simulink model "Copy_of_NDI"  (R2024b)
settings: Solver=ode4  StartTime=0  StopTime=100  FixedStep=fcs.Ts  RelTol=1e-3
PreLoadFcn:
  | FlightPhase = 'FallingLeaf';
  | % FlightPhase = 'InAir';
  | % FlightPhase = 'TVC_h10000V617alpha2';
  | run('PreLoadFcn.m')
values from neighbouring files (symbols this model uses):
  ControlAllocation = 1    [PreLoadFcn.m]    (also in RunThis_ChiaWei.m = 4; RunThis_LM.m = 4; RunThis_Shao.m; RunThis_james.m = 10)
  DUmax = IN_MAT(k+4,1:m)'    [LP_def.m]    (also in LP_lift.m; LP_sig.m; LP_thrust.m; PreLoadFcn.m = [Aactuator.right_aileron.RateLimitUpper Aactuator.left_ailer)
  DUmin = IN_MAT(k+5,1:m)'    [LP_def.m]    (also in LP_lift.m; LP_sig.m; LP_thrust.m; PreLoadFcn.m = [Aactuator.right_aileron.RateLimitLower Aactuator.left_ailer)
  g = [ 0  0  32.17 ]    [PreLoadFcn.m]
  hground = 0    [PreLoadFcn.m]
  m = m1-1    [CGIwrap.m]    (also in DAISY_CHAINING.m; DA_Allocation.m; LP_BasicSolution.m; LP_def.m)
  Mode_deflection_aileron = 1    [PreLoadFcn.m]    (also in RunThis_ChiaWei.m; RunThis_Shao.m = 0)
  Mode_deflection_elevator = 1    [PreLoadFcn.m]    (also in RunThis_ChiaWei.m; RunThis_Shao.m = 0)
  Mode_deflection_rudder = 1    [PreLoadFcn.m]    (also in RunThis_ChiaWei.m; RunThis_Shao.m = 0)
  Mode_deflection_TVC_y = 1    [PreLoadFcn.m]    (also in RunThis_ChiaWei.m; RunThis_Shao.m = 2)
  Mode_deflection_TVC_z = 1    [PreLoadFcn.m]    (also in RunThis_ChiaWei.m; RunThis_Shao.m = 0)
  N = IN_MAT(k+7:k+15,1:m)    [CGIwrap.m]    (also in DAISY_CHAINING.m; PreLoadFcn.m = [ 1      0     0.25; RunThis_ChiaWei.m = [ 1      0     0.25; RunThis_LM.m = [ 1      0     0.25)
  Ninv_2nozzle = inv(diag([  1/21.5  1/21.5  1/25  1/25  1/30  1/15  1/15  1/15  1/15 ]))    [PreLoadFcn.m]
  Ninv_no_nozzle = diag([    21.5    21.5    25    25    30    0     0     0     0  ])    [PreLoadFcn.m]
  state0 = [IC.npos IC.epos IC.alt IC.q0 IC.q1 IC.q2 IC.q3  IC.p IC.q IC.r IC.alpha IC.beta IC.mu IC.Vt IC.chi IC.gamma]    [PreLoadFcn.m]
  Umax_2nozzle = [Aactuator.right_aileron.AngleLimitUpper  Aactuator.left_aileron.AngleLimitUpper  Aactuator.right_elevator.AngleLimitUpper Aactuator.left_elevator.AngleLimitUpper  Aactuator.rudder.AngleLimitUpper                  Aactuator.TVC_ry.AngleLimitUpper    Aactuator.TVC_rz.AngleLimitUpper  Aactuator.TVC_ly.AngleLimitUpper    Aactuator.TVC_lz.AngleLimitUpper]    [PreLoadFcn.m]
  Umax_no_nozzle = [Aactuator.right_aileron.AngleLimitUpper  Aactuator.left_aileron.AngleLimitUpper  Aactuator.right_elevator.AngleLimitUpper Aactuator.left_elevator.AngleLimitUpper  Aactuator.rudder.AngleLimitUpper                    0 0 0 0]    [PreLoadFcn.m]
  Umin_2nozzle = [Aactuator.aileron.AngleLimitLower  Aactuator.aileron.AngleLimitLower  Aactuator.elevator.AngleLimitLower Aactuator.elevator.AngleLimitLower  Aactuator.rudder.AngleLimitLower                  Aactuator.TVC_ry.AngleLimitLower    Aactuator.TVC_rz.AngleLimitLower Aactuator.TVC_ly.AngleLimitLower    Aactuator.TVC_lz.AngleLimitLower]    [PreLoadFcn.m]
  Umin_no_nozzle = [Aactuator.right_aileron.AngleLimitLower  Aactuator.left_aileron.AngleLimitLower  Aactuator.right_elevator.AngleLimitLower Aactuator.left_elevator.AngleLimitLower  Aactuator.rudder.AngleLimitLower                    0 0 0 0]    [PreLoadFcn.m]
undefined symbols (not defined in the file or in its folder): Aactuator, ac, AeroCoeff, EngineTable, F, fcs, ft, IC, kg, LandingGear, Light, MIL, PIController, s, Sensor, sigbuilder_block, slug, sysID_DAQ, sysID_OBES, WMM2020
libraries: aerolibconvert2 x31, slpidlib x11, simulink x6, sharedutil x4, aerolibatmos2 x3, aerolibwind2 x3, aerolibbdyn x3, aerolibgravity2 x2, sharedtransform x1
(part 6 of 14)

== system Copy_of_NDI/F-16 Vehicle Systems Model/Pilot commands storehouse/trun(deg) 初始高度10000ft 初始速度100ft//s攻角30度 ==
  Demux : Demux  Tag=STV Demux  Outputs=5
      settings: DisplayOption=none
  FromWs : FromWorkspace  Tag=STV FromWs  VariableName=tuvar
      SigBuilderData=|
      | common.afterFinalStr = 'Extrapolate'
      | common.sampleTime = 0
      | dataSet.timeRange = [0 20]
      | dataSet.name = 'Group 5'
      | sbobj.Groups.Name = 'Group 5'
      | sbobj.Groups.Signals(1).Name = 'mu'
      | sbobj.Groups.Signals(1).XData = [0 2 5.5 6.5 8.2 9.5 10 13 15 20]
      | sbobj.Groups.Signals(1).YData = [0 0 0 -80 -120 -120 -120 -70 -40 -10]
      | sbobj.Groups.Signals(2).Name = 'alpha'
      | sbobj.Groups.Signals(2).XData = [0 4 7.8 9.2 12.5 14 16 20]
      | sbobj.Groups.Signals(2).YData = [5 5 30 30 10 5 5 5]
      | sbobj.Groups.Signals(3).Name = 'beta'
      | sbobj.Groups.Signals(3).XData = [0 20]
      | sbobj.Groups.Signals(3).YData = [0 0]
      | sbobj.Groups.Signals(4).Name = 'speed brake'
      | sbobj.Groups.Signals(4).XData = [0 20]
      | sbobj.Groups.Signals(4).YData = [0 0]
      | sbobj.Groups.Signals(5).Name = 'LandingGear_down'
      | sbobj.Groups.Signals(5).XData = [0 20]
      | sbobj.Groups.Signals(5).YData = [1 1]
      | sbobj.Groups.TimeRange = [0 20]
  mu : Outport  Tag=STV Outport  VectorParamsAs1DForOutWhenUnconnected=off
  alpha : Outport  Tag=STV Outport  Port=2  VectorParamsAs1DForOutWhenUnconnected=off
  beta : Outport  Tag=STV Outport  Port=3  VectorParamsAs1DForOutWhenUnconnected=off
  speed brake : Outport  Tag=STV Outport  Port=4
  LandingGear_down : Outport  Tag=STV Outport  Port=5
  wires:
  Demux/5 -> LandingGear_down/1
  Demux/4 -> speed brake/1
  Demux/3 -> beta/1
  Demux/2 -> alpha/1
  Demux/1 -> mu/1
  FromWs/1 -> Demux/1

== system Copy_of_NDI/F-16 Vehicle Systems Model/Pilot commands storehouse/trun(deg) 初始高度10000ft 初始速度150ft//s攻角40度1 ==
  Demux : Demux  Tag=STV Demux  Outputs=5
      settings: DisplayOption=none
  FromWs : FromWorkspace  Tag=STV FromWs  VariableName=tuvar
      SigBuilderData=|
      | common.afterFinalStr = 'Extrapolate'
      | common.sampleTime = 0
      | dataSet.timeRange = [0 20]
      | dataSet.name = 'Group 5'
      | sbobj.Groups.Name = 'Group 5'
      | sbobj.Groups.Signals(1).Name = 'mu'
      | sbobj.Groups.Signals(1).XData = [0 2 5.5 7 8.7 10 11 13 15 20]
      | sbobj.Groups.Signals(1).YData = [0 0 -19.5 -60 -150 -150 -150 -70 -40 -10]
      | sbobj.Groups.Signals(2).Name = 'alpha'
      | sbobj.Groups.Signals(2).XData = [0 5 7.8 8.2 10 12.5 14 20]
      | sbobj.Groups.Signals(2).YData = [7 10 40 40 20 10.68 10 10]
      | sbobj.Groups.Signals(3).Name = 'beta'
      | sbobj.Groups.Signals(3).XData = [0 20]
      | sbobj.Groups.Signals(3).YData = [0 0]
      | sbobj.Groups.Signals(4).Name = 'speed brake'
      | sbobj.Groups.Signals(4).XData = [0 20]
      | sbobj.Groups.Signals(4).YData = [0 0]
      | sbobj.Groups.Signals(5).Name = 'LandingGear_down'
      | sbobj.Groups.Signals(5).XData = [0 20]
      | sbobj.Groups.Signals(5).YData = [1 1]
      | sbobj.Groups.TimeRange = [0 20]
  mu : Outport  Tag=STV Outport  VectorParamsAs1DForOutWhenUnconnected=off
  alpha : Outport  Tag=STV Outport  Port=2  VectorParamsAs1DForOutWhenUnconnected=off
  beta : Outport  Tag=STV Outport  Port=3  VectorParamsAs1DForOutWhenUnconnected=off
  speed brake : Outport  Tag=STV Outport  Port=4
  LandingGear_down : Outport  Tag=STV Outport  Port=5
  wires:
  Demux/5 -> LandingGear_down/1
  Demux/4 -> speed brake/1
  Demux/3 -> beta/1
  Demux/2 -> alpha/1
  Demux/1 -> mu/1
  FromWs/1 -> Demux/1

== system Copy_of_NDI/F-16 Vehicle Systems Model/Pilot commands storehouse/trun(deg) 初始高度10000ft 初始速度250ft//s攻角40度1 ==
  Demux : Demux  Tag=STV Demux  Outputs=5
      settings: DisplayOption=none
  FromWs : FromWorkspace  Tag=STV FromWs  VariableName=tuvar
      SigBuilderData=|
      | common.afterFinalStr = 'Extrapolate'
      | common.sampleTime = 0
      | dataSet.timeRange = [0 20]
      | dataSet.name = 'Group 5'
      | sbobj.Groups.Name = 'Group 5'
      | sbobj.Groups.Signals(1).Name = 'mu'
      | sbobj.Groups.Signals(1).XData = [0 2 5.5 7 8.7 8.7 10 11 13 15 20]
      | sbobj.Groups.Signals(1).YData = [0 0 -19.5 -122 -172 -170 -170 -170 -70 -40 -10]
      | sbobj.Groups.Signals(2).Name = 'alpha'
      | sbobj.Groups.Signals(2).XData = [0 5 7.8 8.2 10 12.5 14 20]
      | sbobj.Groups.Signals(2).YData = [7 10 40 40 20 10.68 10 10]
      | sbobj.Groups.Signals(3).Name = 'beta'
      | sbobj.Groups.Signals(3).XData = [0 20]
      | sbobj.Groups.Signals(3).YData = [0 0]
      | sbobj.Groups.Signals(4).Name = 'speed brake'
      | sbobj.Groups.Signals(4).XData = [0 20]
      | sbobj.Groups.Signals(4).YData = [0 0]
      | sbobj.Groups.Signals(5).Name = 'LandingGear_down'
      | sbobj.Groups.Signals(5).XData = [0 20]
      | sbobj.Groups.Signals(5).YData = [1 1]
      | sbobj.Groups.TimeRange = [0 20]
  mu : Outport  Tag=STV Outport  VectorParamsAs1DForOutWhenUnconnected=off
  alpha : Outport  Tag=STV Outport  Port=2  VectorParamsAs1DForOutWhenUnconnected=off
  beta : Outport  Tag=STV Outport  Port=3  VectorParamsAs1DForOutWhenUnconnected=off
  speed brake : Outport  Tag=STV Outport  Port=4
  LandingGear_down : Outport  Tag=STV Outport  Port=5
  wires:
  Demux/5 -> LandingGear_down/1
  Demux/4 -> speed brake/1
  Demux/3 -> beta/1
  Demux/2 -> alpha/1
  Demux/1 -> mu/1
  FromWs/1 -> Demux/1

== system Copy_of_NDI/F-16 Vehicle Systems Model/Pilot commands storehouse/trun(deg) 初始高度10000ft 初始速度350ft//s攻角40度 ==
  Demux : Demux  Tag=STV Demux  Outputs=5
      settings: DisplayOption=none
  FromWs : FromWorkspace  Tag=STV FromWs  VariableName=tuvar
      SigBuilderData=|
      | common.afterFinalStr = 'Extrapolate'
      | common.sampleTime = 0
      | dataSet.timeRange = [0 20]
      | dataSet.name = 'Group 5'
      | sbobj.Groups.Name = 'Group 5'
      | sbobj.Groups.Signals(1).Name = 'mu'
      | sbobj.Groups.Signals(1).XData = [0 2 5.5 6.5 8.2 10 11 13 15 20]
      | sbobj.Groups.Signals(1).YData = [0 0 -19.5 -122 -170 -170 -170 -70 -40 -10]
      | sbobj.Groups.Signals(2).Name = 'alpha'
      | sbobj.Groups.Signals(2).XData = [0 5 7.8 8.2 10 12.5 14 20]
      | sbobj.Groups.Signals(2).YData = [7 10 40 40 20 10.68 10 10]
      | sbobj.Groups.Signals(3).Name = 'beta'
      | sbobj.Groups.Signals(3).XData = [0 20]
      | sbobj.Groups.Signals(3).YData = [0 0]
      | sbobj.Groups.Signals(4).Name = 'speed brake'
      | sbobj.Groups.Signals(4).XData = [0 20]
      | sbobj.Groups.Signals(4).YData = [0 0]
      | sbobj.Groups.Signals(5).Name = 'LandingGear_down'
      | sbobj.Groups.Signals(5).XData = [0 20]
      | sbobj.Groups.Signals(5).YData = [1 1]
      | sbobj.Groups.TimeRange = [0 20]
  mu : Outport  Tag=STV Outport  VectorParamsAs1DForOutWhenUnconnected=off
  alpha : Outport  Tag=STV Outport  Port=2  VectorParamsAs1DForOutWhenUnconnected=off
  beta : Outport  Tag=STV Outport  Port=3  VectorParamsAs1DForOutWhenUnconnected=off
  speed brake : Outport  Tag=STV Outport  Port=4
  LandingGear_down : Outport  Tag=STV Outport  Port=5
  wires:
  Demux/5 -> LandingGear_down/1
  Demux/4 -> speed brake/1
  Demux/3 -> beta/1
  Demux/2 -> alpha/1
  Demux/1 -> mu/1
  FromWs/1 -> Demux/1

== system Copy_of_NDI/F-16 Vehicle Systems Model/Pilot commands storehouse/trun(deg) 初始高度10000ft 初始速度450ft//s攻角40度 ==
  Demux : Demux  Tag=STV Demux  Outputs=5
      settings: DisplayOption=none
  FromWs : FromWorkspace  Tag=STV FromWs  VariableName=tuvar
      SigBuilderData=|
      | common.afterFinalStr = 'Extrapolate'
      | common.sampleTime = 0
      | dataSet.timeRange = [0 20]
      | dataSet.name = 'Group 5'
      | sbobj.Groups.Name = 'Group 5'
      | sbobj.Groups.Signals(1).Name = 'mu'
      | sbobj.Groups.Signals(1).XData = [0 2 5.5 6.5 7.5 8.5 10 12 15 20]
      | sbobj.Groups.Signals(1).YData = [0 0 -19.5 -120 -150 -150 -150 -70 -40 -10]
      | sbobj.Groups.Signals(2).Name = 'alpha'
      | sbobj.Groups.Signals(2).XData = [0 5 7.2 7.8 10 12.5 14 20]
      | sbobj.Groups.Signals(2).YData = [7 10 40 40 20 10.68 10 10]
      | sbobj.Groups.Signals(3).Name = 'beta'
      | sbobj.Groups.Signals(3).XData = [0 20]
      | sbobj.Groups.Signals(3).YData = [0 0]
      | sbobj.Groups.Signals(4).Name = 'speed brake'
      | sbobj.Groups.Signals(4).XData = [0 20]
      | sbobj.Groups.Signals(4).YData = [0 0]
      | sbobj.Groups.Signals(5).Name = 'LandingGear_down'
      | sbobj.Groups.Signals(5).XData = [0 20]
      | sbobj.Groups.Signals(5).YData = [1 1]
      | sbobj.Groups.TimeRange = [0 20]
  mu : Outport  Tag=STV Outport  VectorParamsAs1DForOutWhenUnconnected=off
  alpha : Outport  Tag=STV Outport  Port=2  VectorParamsAs1DForOutWhenUnconnected=off
  beta : Outport  Tag=STV Outport  Port=3  VectorParamsAs1DForOutWhenUnconnected=off
  speed brake : Outport  Tag=STV Outport  Port=4
  LandingGear_down : Outport  Tag=STV Outport  Port=5
  wires:
  Demux/5 -> LandingGear_down/1
  Demux/4 -> speed brake/1
  Demux/3 -> beta/1
  Demux/2 -> alpha/1
  Demux/1 -> mu/1
  FromWs/1 -> Demux/1

== system Copy_of_NDI/F-16 Vehicle Systems Model/Pilot commands storehouse/trun(deg) 初始高度10000ft 初始速度450ft//s攻角40度1 ==
  Demux : Demux  Tag=STV Demux  Outputs=5
      settings: DisplayOption=none
  FromWs : FromWorkspace  Tag=STV FromWs  VariableName=tuvar
      SigBuilderData=|
      | common.afterFinalStr = 'Extrapolate'
      | common.sampleTime = 0
      | dataSet.timeRange = [0 20]
      | dataSet.name = 'Group 5'
      | sbobj.Groups.Name = 'Group 5'
      | sbobj.Groups.Signals(1).Name = 'mu'
      | sbobj.Groups.Signals(1).XData = [0 2 5.5 6.5 7.5 8.5 10 12 15 20]
      | sbobj.Groups.Signals(1).YData = [0 0 -19.5 -120 -150 -150 -150 -70 -40 -10]
      | sbobj.Groups.Signals(2).Name = 'alpha'
      | sbobj.Groups.Signals(2).XData = [0 5 7.2 7.8 10 12.5 14 20]
      | sbobj.Groups.Signals(2).YData = [7 10 40 40 20 10.68 10 10]
      | sbobj.Groups.Signals(3).Name = 'beta'
      | sbobj.Groups.Signals(3).XData = [0 20]
      | sbobj.Groups.Signals(3).YData = [0 0]
      | sbobj.Groups.Signals(4).Name = 'speed brake'
      | sbobj.Groups.Signals(4).XData = [0 20]
      | sbobj.Groups.Signals(4).YData = [0 0]
      | sbobj.Groups.Signals(5).Name = 'LandingGear_down'
      | sbobj.Groups.Signals(5).XData = [0 20]
      | sbobj.Groups.Signals(5).YData = [1 1]
      | sbobj.Groups.TimeRange = [0 20]
  mu : Outport  Tag=STV Outport  VectorParamsAs1DForOutWhenUnconnected=off
  alpha : Outport  Tag=STV Outport  Port=2  VectorParamsAs1DForOutWhenUnconnected=off
  beta : Outport  Tag=STV Outport  Port=3  VectorParamsAs1DForOutWhenUnconnected=off
  speed brake : Outport  Tag=STV Outport  Port=4
  LandingGear_down : Outport  Tag=STV Outport  Port=5
  wires:
  Demux/5 -> LandingGear_down/1
  Demux/4 -> speed brake/1
  Demux/3 -> beta/1
  Demux/2 -> alpha/1
  Demux/1 -> mu/1
  FromWs/1 -> Demux/1

== system Copy_of_NDI/F-16 Vehicle Systems Model/Pilot commands storehouse/trun(deg) 初始高度10000ft 初始速度500ft//s攻角30度1 ==
  Demux : Demux  Tag=STV Demux  Outputs=5
      settings: DisplayOption=none
  FromWs : FromWorkspace  Tag=STV FromWs  VariableName=tuvar
      SigBuilderData=|
      | common.afterFinalStr = 'Extrapolate'
      | common.sampleTime = 0
      | dataSet.timeRange = [0 20]
      | dataSet.name = 'Group 5'
      | sbobj.Groups.Name = 'Group 5'
      | sbobj.Groups.Signals(1).Name = 'mu'
      | sbobj.Groups.Signals(1).XData = [0 2 5.5 6.7 8.2 9.5 10 13 15 20]
      | sbobj.Groups.Signals(1).YData = [0 0 20 -80 -120 -120 -120 -70 -40 -10]
      | sbobj.Groups.Signals(2).Name = 'alpha'
      | sbobj.Groups.Signals(2).XData = [0 2 5.8 9.2 12.5 14 16 20]
      | sbobj.Groups.Signals(2).YData = [5 5 30 30 10 5 5 5]
      | sbobj.Groups.Signals(3).Name = 'beta'
      | sbobj.Groups.Signals(3).XData = [0 20]
      | sbobj.Groups.Signals(3).YData = [0 0]
      | sbobj.Groups.Signals(4).Name = 'speed brake'
      | sbobj.Groups.Signals(4).XData = [0 20]
      | sbobj.Groups.Signals(4).YData = [0 0]
      | sbobj.Groups.Signals(5).Name = 'LandingGear_down'
      | sbobj.Groups.Signals(5).XData = [0 20]
      | sbobj.Groups.Signals(5).YData = [1 1]
      | sbobj.Groups.TimeRange = [0 20]
  mu : Outport  Tag=STV Outport  VectorParamsAs1DForOutWhenUnconnected=off
  alpha : Outport  Tag=STV Outport  Port=2  VectorParamsAs1DForOutWhenUnconnected=off
  beta : Outport  Tag=STV Outport  Port=3  VectorParamsAs1DForOutWhenUnconnected=off
  speed brake : Outport  Tag=STV Outport  Port=4
  LandingGear_down : Outport  Tag=STV Outport  Port=5
  wires:
  Demux/5 -> LandingGear_down/1
  Demux/4 -> speed brake/1
  Demux/3 -> beta/1
  Demux/2 -> alpha/1
  Demux/1 -> mu/1
  FromWs/1 -> Demux/1

== system Copy_of_NDI/F-16 Vehicle Systems Model/Pilot commands storehouse/trun(deg) 初始高度10000ft 初始速度550ft//s攻角40度 ==
  Demux : Demux  Tag=STV Demux  Outputs=5
      settings: DisplayOption=none
  FromWs : FromWorkspace  Tag=STV FromWs  VariableName=tuvar
      SigBuilderData=|
      | common.afterFinalStr = 'Extrapolate'
      | common.sampleTime = 0
      | dataSet.timeRange = [0 20]
      | dataSet.name = 'Group 5'
      | sbobj.Groups.Name = 'Group 5'
      | sbobj.Groups.Signals(1).Name = 'mu'
      | sbobj.Groups.Signals(1).XData = [0 2 5.5 6 7.2 8.5 10 12 15 20]
      | sbobj.Groups.Signals(1).YData = [0 0 -19.5 -120 -150 -150 -150 -70 -40 -10]
      | sbobj.Groups.Signals(2).Name = 'alpha'
      | sbobj.Groups.Signals(2).XData = [0 5 7.2 7.8 10 12.5 14 20]
      | sbobj.Groups.Signals(2).YData = [7 10 40 40 20 10.68 10 10]
      | sbobj.Groups.Signals(3).Name = 'beta'
      | sbobj.Groups.Signals(3).XData = [0 20]
      | sbobj.Groups.Signals(3).YData = [0 0]
      | sbobj.Groups.Signals(4).Name = 'speed brake'
      | sbobj.Groups.Signals(4).XData = [0 20]
      | sbobj.Groups.Signals(4).YData = [0 0]
      | sbobj.Groups.Signals(5).Name = 'LandingGear_down'
      | sbobj.Groups.Signals(5).XData = [0 20]
      | sbobj.Groups.Signals(5).YData = [1 1]
      | sbobj.Groups.TimeRange = [0 20]
  mu : Outport  Tag=STV Outport  VectorParamsAs1DForOutWhenUnconnected=off
  alpha : Outport  Tag=STV Outport  Port=2  VectorParamsAs1DForOutWhenUnconnected=off
  beta : Outport  Tag=STV Outport  Port=3  VectorParamsAs1DForOutWhenUnconnected=off
  speed brake : Outport  Tag=STV Outport  Port=4
  LandingGear_down : Outport  Tag=STV Outport  Port=5
  wires:
  Demux/5 -> LandingGear_down/1
  Demux/4 -> speed brake/1
  Demux/3 -> beta/1
  Demux/2 -> alpha/1
  Demux/1 -> mu/1
  FromWs/1 -> Demux/1

== system Copy_of_NDI/F-16 Vehicle Systems Model/Pilot commands storehouse/trun(deg) 初始高度10000ft 初始速度550ft//s攻角40度1 ==
  Demux : Demux  Tag=STV Demux  Outputs=5
      settings: DisplayOption=none
  FromWs : FromWorkspace  Tag=STV FromWs  VariableName=tuvar
      SigBuilderData=|
      | common.afterFinalStr = 'Extrapolate'
      | common.sampleTime = 0
      | dataSet.timeRange = [0 20]
      | dataSet.name = 'Group 5'
      | sbobj.Groups.Name = 'Group 5'
      | sbobj.Groups.Signals(1).Name = 'mu'
      | sbobj.Groups.Signals(1).XData = [0 2 5.5 6 7.2 8.5 10 12 15 20]
      | sbobj.Groups.Signals(1).YData = [0 0 -19.5 -120 -150 -150 -150 -70 -40 -10]
      | sbobj.Groups.Signals(2).Name = 'alpha'
      | sbobj.Groups.Signals(2).XData = [0 5 7.2 7.8 10 12.5 14 20]
      | sbobj.Groups.Signals(2).YData = [7 10 40 40 20 10.68 10 10]
      | sbobj.Groups.Signals(3).Name = 'beta'
      | sbobj.Groups.Signals(3).XData = [0 20]
      | sbobj.Groups.Signals(3).YData = [0 0]
      | sbobj.Groups.Signals(4).Name = 'speed brake'
      | sbobj.Groups.Signals(4).XData = [0 20]
      | sbobj.Groups.Signals(4).YData = [0 0]
      | sbobj.Groups.Signals(5).Name = 'LandingGear_down'
      | sbobj.Groups.Signals(5).XData = [0 20]
      | sbobj.Groups.Signals(5).YData = [1 1]
      | sbobj.Groups.TimeRange = [0 20]
  mu : Outport  Tag=STV Outport  VectorParamsAs1DForOutWhenUnconnected=off
  alpha : Outport  Tag=STV Outport  Port=2  VectorParamsAs1DForOutWhenUnconnected=off
  beta : Outport  Tag=STV Outport  Port=3  VectorParamsAs1DForOutWhenUnconnected=off
  speed brake : Outport  Tag=STV Outport  Port=4
  LandingGear_down : Outport  Tag=STV Outport  Port=5
  wires:
  Demux/5 -> LandingGear_down/1
  Demux/4 -> speed brake/1
  Demux/3 -> beta/1
  Demux/2 -> alpha/1
  Demux/1 -> mu/1
  FromWs/1 -> Demux/1

== system Copy_of_NDI/F-16 Vehicle Systems Model/Pilot commands storehouse/trun(deg) 初始高度10000ft 初始速度650ft//s攻角40度1 ==
  Demux : Demux  Tag=STV Demux  Outputs=5
      settings: DisplayOption=none
  FromWs : FromWorkspace  Tag=STV FromWs  VariableName=tuvar
      SigBuilderData=|
      | common.afterFinalStr = 'Extrapolate'
      | common.sampleTime = 0
      | dataSet.timeRange = [0 20]
      | dataSet.name = 'Group 5'
      | sbobj.Groups.Name = 'Group 5'
      | sbobj.Groups.Signals(1).Name = 'mu'
      | sbobj.Groups.Signals(1).XData = [0 2 5.5 6 7.2 8.5 10 12 15 20]
      | sbobj.Groups.Signals(1).YData = [0 0 -10 -140 -160 -160 -150 -70 -40 -10]
      | sbobj.Groups.Signals(2).Name = 'alpha'
      | sbobj.Groups.Signals(2).XData = [0 5 7.2 7.8 10 12.5 14 20]
      | sbobj.Groups.Signals(2).YData = [7 10 40 40 20 10.68 10 10]
      | sbobj.Groups.Signals(3).Name = 'beta'
      | sbobj.Groups.Signals(3).XData = [0 20]
      | sbobj.Groups.Signals(3).YData = [0 0]
      | sbobj.Groups.Signals(4).Name = 'speed brake'
      | sbobj.Groups.Signals(4).XData = [0 20]
      | sbobj.Groups.Signals(4).YData = [0 0]
      | sbobj.Groups.Signals(5).Name = 'LandingGear_down'
      | sbobj.Groups.Signals(5).XData = [0 20]
      | sbobj.Groups.Signals(5).YData = [1 1]
      | sbobj.Groups.TimeRange = [0 20]
  mu : Outport  Tag=STV Outport  VectorParamsAs1DForOutWhenUnconnected=off
  alpha : Outport  Tag=STV Outport  Port=2  VectorParamsAs1DForOutWhenUnconnected=off
  beta : Outport  Tag=STV Outport  Port=3  VectorParamsAs1DForOutWhenUnconnected=off
  speed brake : Outport  Tag=STV Outport  Port=4
  LandingGear_down : Outport  Tag=STV Outport  Port=5
  wires:
  Demux/5 -> LandingGear_down/1
  Demux/4 -> speed brake/1
  Demux/3 -> beta/1
  Demux/2 -> alpha/1
  Demux/1 -> mu/1
  FromWs/1 -> Demux/1

== system Copy_of_NDI/F-16 Vehicle Systems Model/Pilot commands storehouse/trun(deg) 初始高度10000ft 初始速度750ft//s攻角40度 ==
  Demux : Demux  Tag=STV Demux  Outputs=5
      settings: DisplayOption=none
  FromWs : FromWorkspace  Tag=STV FromWs  VariableName=tuvar
      SigBuilderData=|
      | common.afterFinalStr = 'Extrapolate'
      | common.sampleTime = 0
      | dataSet.timeRange = [0 20]
      | dataSet.name = 'Group 5'
      | sbobj.Groups.Name = 'Group 5'
      | sbobj.Groups.Signals(1).Name = 'mu'
      | sbobj.Groups.Signals(1).XData = [0 2 5.5 6 7.2 8.5 10 12 15 20]
      | sbobj.Groups.Signals(1).YData = [0 0 0 -150 -170 -170 -160 -70 -40 -10]
      | sbobj.Groups.Signals(2).Name = 'alpha'
      | sbobj.Groups.Signals(2).XData = [0 5 7.2 7.8 10 12.5 14 20]
      | sbobj.Groups.Signals(2).YData = [7 10 40 40 20 10.68 10 10]
      | sbobj.Groups.Signals(3).Name = 'beta'
      | sbobj.Groups.Signals(3).XData = [0 20]
      | sbobj.Groups.Signals(3).YData = [0 0]
      | sbobj.Groups.Signals(4).Name = 'speed brake'
      | sbobj.Groups.Signals(4).XData = [0 20]
      | sbobj.Groups.Signals(4).YData = [0 0]
      | sbobj.Groups.Signals(5).Name = 'LandingGear_down'
      | sbobj.Groups.Signals(5).XData = [0 20]
      | sbobj.Groups.Signals(5).YData = [1 1]
      | sbobj.Groups.TimeRange = [0 20]
  mu : Outport  Tag=STV Outport  VectorParamsAs1DForOutWhenUnconnected=off
  alpha : Outport  Tag=STV Outport  Port=2  VectorParamsAs1DForOutWhenUnconnected=off
  beta : Outport  Tag=STV Outport  Port=3  VectorParamsAs1DForOutWhenUnconnected=off
  speed brake : Outport  Tag=STV Outport  Port=4
  LandingGear_down : Outport  Tag=STV Outport  Port=5
  wires:
  Demux/5 -> LandingGear_down/1
  Demux/4 -> speed brake/1
  Demux/3 -> beta/1
  Demux/2 -> alpha/1
  Demux/1 -> mu/1
  FromWs/1 -> Demux/1

== system Copy_of_NDI/F-16 Vehicle Systems Model/Pilot commands storehouse/trun(deg)非高攻角 初始高度10000ft 初始速度250ft//s ==
  Demux : Demux  Tag=STV Demux  Outputs=5
      settings: DisplayOption=none
  FromWs : FromWorkspace  Tag=STV FromWs  VariableName=tuvar
      SigBuilderData=|
      | common.afterFinalStr = 'Extrapolate'
      | common.sampleTime = 0
      | dataSet.timeRange = [0 20]
      | dataSet.name = 'Group 5'
      | sbobj.Groups.Name = 'Group 5'
      | sbobj.Groups.Signals(1).Name = 'mu'
      | sbobj.Groups.Signals(1).XData = [0 2 5.5 7 8.7 10.4 11.9 15 20]
      | sbobj.Groups.Signals(1).YData = [0 20.6 -19.5 -120 -160 -120 -40.1 -20 -10]
      | sbobj.Groups.Signals(2).Name = 'alpha'
      | sbobj.Groups.Signals(2).XData = [0 5 7.8 8.2 10 12.5 14 20]
      | sbobj.Groups.Signals(2).YData = [7 10 40 40 20 10.68 10 10]
      | sbobj.Groups.Signals(3).Name = 'beta'
      | sbobj.Groups.Signals(3).XData = [0 20]
      | sbobj.Groups.Signals(3).YData = [0 0]
      | sbobj.Groups.Signals(4).Name = 'speed brake'
      | sbobj.Groups.Signals(4).XData = [0 20]
      | sbobj.Groups.Signals(4).YData = [0 0]
      | sbobj.Groups.Signals(5).Name = 'LandingGear_down'
      | sbobj.Groups.Signals(5).XData = [0 20]
      | sbobj.Groups.Signals(5).YData = [1 1]
      | sbobj.Groups.TimeRange = [0 20]
  mu : Outport  Tag=STV Outport  VectorParamsAs1DForOutWhenUnconnected=off
  alpha : Outport  Tag=STV Outport  Port=2  VectorParamsAs1DForOutWhenUnconnected=off
  beta : Outport  Tag=STV Outport  Port=3  VectorParamsAs1DForOutWhenUnconnected=off
  speed brake : Outport  Tag=STV Outport  Port=4
  LandingGear_down : Outport  Tag=STV Outport  Port=5
  wires:
  Demux/5 -> LandingGear_down/1
  Demux/4 -> speed brake/1
  Demux/3 -> beta/1
  Demux/2 -> alpha/1
  Demux/1 -> mu/1
  FromWs/1 -> Demux/1

== system Copy_of_NDI/F-16 Vehicle Systems Model/Pilot commands storehouse/trun(deg)非高攻角 初始高度10000ft 初始速度250ft//s(碩論6.2,6.3,7.2) ==
  Demux : Demux  Tag=STV Demux  Outputs=5
      settings: DisplayOption=none
  FromWs : FromWorkspace  Tag=STV FromWs  VariableName=tuvar
      SigBuilderData=|
      | common.afterFinalStr = 'Extrapolate'
      | common.sampleTime = 0
      | dataSet.timeRange = [0 20]
      | dataSet.name = 'Group 5'
      | sbobj.Groups.Name = 'Group 5'
      | sbobj.Groups.Signals(1).Name = 'mu'
      | sbobj.Groups.Signals(1).XData = [0 2 5.5 7 8.7 10.4 11.9 15 20]
      | sbobj.Groups.Signals(1).YData = [0 20.6 -19.5 -120 -160 -120 -100 -47.5 -10]
      | sbobj.Groups.Signals(2).Name = 'alpha'
      | sbobj.Groups.Signals(2).XData = [0 5 7.8 8.2 10 12.5 14 20]
      | sbobj.Groups.Signals(2).YData = [7 10 40 40 20 10.68 10 10]
      | sbobj.Groups.Signals(3).Name = 'beta'
      | sbobj.Groups.Signals(3).XData = [0 20]
      | sbobj.Groups.Signals(3).YData = [0 0]
      | sbobj.Groups.Signals(4).Name = 'speed brake'
      | sbobj.Groups.Signals(4).XData = [0 20]
      | sbobj.Groups.Signals(4).YData = [0 0]
      | sbobj.Groups.Signals(5).Name = 'LandingGear_down'
      | sbobj.Groups.Signals(5).XData = [0 20]
      | sbobj.Groups.Signals(5).YData = [1 1]
      | sbobj.Groups.TimeRange = [0 20]
  mu : Outport  Tag=STV Outport  VectorParamsAs1DForOutWhenUnconnected=off
  alpha : Outport  Tag=STV Outport  Port=2  VectorParamsAs1DForOutWhenUnconnected=off
  beta : Outport  Tag=STV Outport  Port=3  VectorParamsAs1DForOutWhenUnconnected=off
  speed brake : Outport  Tag=STV Outport  Port=4
  LandingGear_down : Outport  Tag=STV Outport  Port=5
  wires:
  Demux/5 -> LandingGear_down/1
  Demux/4 -> speed brake/1
  Demux/3 -> beta/1
  Demux/2 -> alpha/1
  Demux/1 -> mu/1
  FromWs/1 -> Demux/1

== system Copy_of_NDI/F-16 Vehicle Systems Model/Pilot commands storehouse/trun(deg)非高攻角 初始高度10000ft 初始速度250ft//s(碩論6.8.1) ==
  Demux : Demux  Tag=STV Demux  Outputs=5
      settings: DisplayOption=none
  FromWs : FromWorkspace  Tag=STV FromWs  VariableName=tuvar
      SigBuilderData=|
      | common.afterFinalStr = 'Extrapolate'
      | common.sampleTime = 0
      | dataSet.timeRange = [0 20]
      | dataSet.name = 'Group 5'
      | sbobj.Groups.Name = 'Group 5'
      | sbobj.Groups.Signals(1).Name = 'mu'
      | sbobj.Groups.Signals(1).XData = [0 2 5.5 6.5 8.7 9.9 11.9 15 20]
      | sbobj.Groups.Signals(1).YData = [0 20.6 -19.5 -120 -160 -120 -100 -55 -10]
      | sbobj.Groups.Signals(2).Name = 'alpha'
      | sbobj.Groups.Signals(2).XData = [0 5 7.8 8.2 10 12.5 14 20]
      | sbobj.Groups.Signals(2).YData = [7 10 40 40 20 10.68 10 10]
      | sbobj.Groups.Signals(3).Name = 'beta'
      | sbobj.Groups.Signals(3).XData = [0 20]
      | sbobj.Groups.Signals(3).YData = [0 0]
      | sbobj.Groups.Signals(4).Name = 'speed brake'
      | sbobj.Groups.Signals(4).XData = [0 20]
      | sbobj.Groups.Signals(4).YData = [0 0]
      | sbobj.Groups.Signals(5).Name = 'LandingGear_down'
      | sbobj.Groups.Signals(5).XData = [0 20]
      | sbobj.Groups.Signals(5).YData = [1 1]
      | sbobj.Groups.TimeRange = [0 20]
  mu : Outport  Tag=STV Outport  VectorParamsAs1DForOutWhenUnconnected=off
  alpha : Outport  Tag=STV Outport  Port=2  VectorParamsAs1DForOutWhenUnconnected=off
  beta : Outport  Tag=STV Outport  Port=3  VectorParamsAs1DForOutWhenUnconnected=off
  speed brake : Outport  Tag=STV Outport  Port=4
  LandingGear_down : Outport  Tag=STV Outport  Port=5
  wires:
  Demux/5 -> LandingGear_down/1
  Demux/4 -> speed brake/1
  Demux/3 -> beta/1
  Demux/2 -> alpha/1
  Demux/1 -> mu/1
  FromWs/1 -> Demux/1

== system Copy_of_NDI/F-16 Vehicle Systems Model/Pilot commands storehouse/trun(deg)非高攻角 初始高度10000ft 初始速度250ft//s(碩論6.8.1)更正 ==
  Demux : Demux  Tag=STV Demux  Outputs=5
      settings: DisplayOption=none
  FromWs : FromWorkspace  Tag=STV FromWs  VariableName=tuvar
      SigBuilderData=|
      | common.afterFinalStr = 'Extrapolate'
      | common.sampleTime = 0
      | dataSet.timeRange = [0 20]
      | dataSet.name = 'Group 5'
      | sbobj.Groups.Name = 'Group 5'
      | sbobj.Groups.Signals(1).Name = 'mu'
      | sbobj.Groups.Signals(1).XData = [0 2 5.5 7 8.7 10.4 11.9 15 20]
      | sbobj.Groups.Signals(1).YData = [0 20.6 -19.5 -140 -160 -120 -100 -65 -10]
      | sbobj.Groups.Signals(2).Name = 'alpha'
      | sbobj.Groups.Signals(2).XData = [0 5 7.8 8.2 10 12.5 14 20]
      | sbobj.Groups.Signals(2).YData = [7 10 40 40 20 10.68 10 10]
      | sbobj.Groups.Signals(3).Name = 'beta'
      | sbobj.Groups.Signals(3).XData = [0 20]
      | sbobj.Groups.Signals(3).YData = [0 0]
      | sbobj.Groups.Signals(4).Name = 'speed brake'
      | sbobj.Groups.Signals(4).XData = [0 20]
      | sbobj.Groups.Signals(4).YData = [0 0]
      | sbobj.Groups.Signals(5).Name = 'LandingGear_down'
      | sbobj.Groups.Signals(5).XData = [0 20]
      | sbobj.Groups.Signals(5).YData = [1 1]
      | sbobj.Groups.TimeRange = [0 20]
  mu : Outport  Tag=STV Outport  VectorParamsAs1DForOutWhenUnconnected=off
  alpha : Outport  Tag=STV Outport  Port=2  VectorParamsAs1DForOutWhenUnconnected=off
  beta : Outport  Tag=STV Outport  Port=3  VectorParamsAs1DForOutWhenUnconnected=off
  speed brake : Outport  Tag=STV Outport  Port=4
  LandingGear_down : Outport  Tag=STV Outport  Port=5
  wires:
  Demux/5 -> LandingGear_down/1
  Demux/4 -> speed brake/1
  Demux/3 -> beta/1
  Demux/2 -> alpha/1
  Demux/1 -> mu/1
  FromWs/1 -> Demux/1

== system Copy_of_NDI/F-16 Vehicle Systems Model/Pilot commands storehouse/trun(deg)非高攻角 初始高度10000ft 初始速度500 600ft//s攻角60度1 ==
  Demux : Demux  Tag=STV Demux  Outputs=5
      settings: DisplayOption=none
  FromWs : FromWorkspace  Tag=STV FromWs  VariableName=tuvar
      SigBuilderData=|
      | common.afterFinalStr = 'Extrapolate'
      | common.sampleTime = 0
      | dataSet.timeRange = [0 20]
      | dataSet.name = 'Group 5'
      | sbobj.Groups.Name = 'Group 5'
      | sbobj.Groups.Signals(1).Name = 'mu'
      | sbobj.Groups.Signals(1).XData = [0 2 5 6 7.2 8.5 10 12 15 20]
      | sbobj.Groups.Signals(1).YData = [0 0 -19.5 -120 -150 -150 -150 -70 -40 -10]
      | sbobj.Groups.Signals(2).Name = 'alpha'
      | sbobj.Groups.Signals(2).XData = [0 5 7.2 7.8 10 12.5 14 20]
      | sbobj.Groups.Signals(2).YData = [7 10 60 60 20 10.68 10 10]
      | sbobj.Groups.Signals(3).Name = 'beta'
      | sbobj.Groups.Signals(3).XData = [0 20]
      | sbobj.Groups.Signals(3).YData = [0 0]
      | sbobj.Groups.Signals(4).Name = 'speed brake'
      | sbobj.Groups.Signals(4).XData = [0 20]
      | sbobj.Groups.Signals(4).YData = [0 0]
      | sbobj.Groups.Signals(5).Name = 'LandingGear_down'
      | sbobj.Groups.Signals(5).XData = [0 20]
      | sbobj.Groups.Signals(5).YData = [1 1]
      | sbobj.Groups.TimeRange = [0 20]
  mu : Outport  Tag=STV Outport  VectorParamsAs1DForOutWhenUnconnected=off
  alpha : Outport  Tag=STV Outport  Port=2  VectorParamsAs1DForOutWhenUnconnected=off
  beta : Outport  Tag=STV Outport  Port=3  VectorParamsAs1DForOutWhenUnconnected=off
  speed brake : Outport  Tag=STV Outport  Port=4
  LandingGear_down : Outport  Tag=STV Outport  Port=5
  wires:
  Demux/5 -> LandingGear_down/1
  Demux/4 -> speed brake/1
  Demux/3 -> beta/1
  Demux/2 -> alpha/1
  Demux/1 -> mu/1
  FromWs/1 -> Demux/1

== system Copy_of_NDI/F-16 Vehicle Systems Model/Pilot commands storehouse/trun(deg)非高攻角 初始高度10000ft 初始速度500 600ft//s攻角60度2 ==
  Demux : Demux  Tag=STV Demux  Outputs=5
      settings: DisplayOption=none
  FromWs : FromWorkspace  Tag=STV FromWs  VariableName=tuvar
      SigBuilderData=|
      | common.afterFinalStr = 'Extrapolate'
      | common.sampleTime = 0
      | dataSet.timeRange = [0 20]
      | dataSet.name = 'Group 5'
      | sbobj.Groups.Name = 'Group 5'
      | sbobj.Groups.Signals(1).Name = 'mu'
      | sbobj.Groups.Signals(1).XData = [0 2 5 6 7.2 8.5 10 12 15 20]
      | sbobj.Groups.Signals(1).YData = [0 0 -19.5 -120 -150 -150 -150 -70 -40 -10]
      | sbobj.Groups.Signals(2).Name = 'alpha'
      | sbobj.Groups.Signals(2).XData = [0 5 7.2 7.8 10 12.5 14 20]
      | sbobj.Groups.Signals(2).YData = [7 10 60 60 20 10.68 10 10]
      | sbobj.Groups.Signals(3).Name = 'beta'
      | sbobj.Groups.Signals(3).XData = [0 20]
      | sbobj.Groups.Signals(3).YData = [0 0]
      | sbobj.Groups.Signals(4).Name = 'speed brake'
      | sbobj.Groups.Signals(4).XData = [0 20]
      | sbobj.Groups.Signals(4).YData = [0 0]
      | sbobj.Groups.Signals(5).Name = 'LandingGear_down'
      | sbobj.Groups.Signals(5).XData = [0 20]
      | sbobj.Groups.Signals(5).YData = [1 1]
      | sbobj.Groups.TimeRange = [0 20]
  mu : Outport  Tag=STV Outport  VectorParamsAs1DForOutWhenUnconnected=off
  alpha : Outport  Tag=STV Outport  Port=2  VectorParamsAs1DForOutWhenUnconnected=off
  beta : Outport  Tag=STV Outport  Port=3  VectorParamsAs1DForOutWhenUnconnected=off
  speed brake : Outport  Tag=STV Outport  Port=4
  LandingGear_down : Outport  Tag=STV Outport  Port=5
  wires:
  Demux/5 -> LandingGear_down/1
  Demux/4 -> speed brake/1
  Demux/3 -> beta/1
  Demux/2 -> alpha/1
  Demux/1 -> mu/1
  FromWs/1 -> Demux/1

== system Copy_of_NDI/F-16 Vehicle Systems Model/Pilot commands storehouse/trun(deg)非高攻角 初始高度10000ft 初始速度500ft//s攻角60度 ==
  Demux : Demux  Tag=STV Demux  Outputs=5
      settings: DisplayOption=none
  FromWs : FromWorkspace  Tag=STV FromWs  VariableName=tuvar
      SigBuilderData=|
      | common.afterFinalStr = 'Extrapolate'
      | common.sampleTime = 0
      | dataSet.timeRange = [0 20]
      | dataSet.name = 'Group 5'
      | sbobj.Groups.Name = 'Group 5'
      | sbobj.Groups.Signals(1).Name = 'mu'
      | sbobj.Groups.Signals(1).XData = [0 2 5 6 7.2 8.5 10 12 15 20]
      | sbobj.Groups.Signals(1).YData = [0 0 -19.5 -120 -150 -150 -150 -70 -40 -10]
      | sbobj.Groups.Signals(2).Name = 'alpha'
      | sbobj.Groups.Signals(2).XData = [0 5 7.2 7.8 10 12.5 14 20]
      | sbobj.Groups.Signals(2).YData = [7 10 60 60 20 10.68 10 10]
      | sbobj.Groups.Signals(3).Name = 'beta'
      | sbobj.Groups.Signals(3).XData = [0 20]
      | sbobj.Groups.Signals(3).YData = [0 0]
      | sbobj.Groups.Signals(4).Name = 'speed brake'
      | sbobj.Groups.Signals(4).XData = [0 20]
      | sbobj.Groups.Signals(4).YData = [0 0]
      | sbobj.Groups.Signals(5).Name = 'LandingGear_down'
      | sbobj.Groups.Signals(5).XData = [0 20]
      | sbobj.Groups.Signals(5).YData = [1 1]
      | sbobj.Groups.TimeRange = [0 20]
  mu : Outport  Tag=STV Outport  VectorParamsAs1DForOutWhenUnconnected=off
  alpha : Outport  Tag=STV Outport  Port=2  VectorParamsAs1DForOutWhenUnconnected=off
  beta : Outport  Tag=STV Outport  Port=3  VectorParamsAs1DForOutWhenUnconnected=off
  speed brake : Outport  Tag=STV Outport  Port=4
  LandingGear_down : Outport  Tag=STV Outport  Port=5
  wires:
  Demux/5 -> LandingGear_down/1
  Demux/4 -> speed brake/1
  Demux/3 -> beta/1
  Demux/2 -> alpha/1
  Demux/1 -> mu/1
  FromWs/1 -> Demux/1

== system Copy_of_NDI/F-16 Vehicle Systems Model/Pilot commands storehouse/trun(deg)非高攻角 初始高度10000ft 初始速度550ft//s600ft//s攻角60度 ==
  Demux : Demux  Tag=STV Demux  Outputs=5
      settings: DisplayOption=none
  FromWs : FromWorkspace  Tag=STV FromWs  VariableName=tuvar
      SigBuilderData=|
      | common.afterFinalStr = 'Extrapolate'
      | common.sampleTime = 0
      | dataSet.timeRange = [0 20]
      | dataSet.name = 'Group 5'
      | sbobj.Groups.Name = 'Group 5'
      | sbobj.Groups.Signals(1).Name = 'mu'
      | sbobj.Groups.Signals(1).XData = [0 2 5 6 7.2 8.5 10 12 15 20]
      | sbobj.Groups.Signals(1).YData = [0 0 -19.5 -120 -150 -150 -150 -70 -40 -10]
      | sbobj.Groups.Signals(2).Name = 'alpha'
      | sbobj.Groups.Signals(2).XData = [0 5 7.2 7.8 10 12.5 14 20]
      | sbobj.Groups.Signals(2).YData = [7 10 60 60 20 10.68 10 10]
      | sbobj.Groups.Signals(3).Name = 'beta'
      | sbobj.Groups.Signals(3).XData = [0 20]
      | sbobj.Groups.Signals(3).YData = [0 0]
      | sbobj.Groups.Signals(4).Name = 'speed brake'
      | sbobj.Groups.Signals(4).XData = [0 20]
      | sbobj.Groups.Signals(4).YData = [0 0]
      | sbobj.Groups.Signals(5).Name = 'LandingGear_down'
      | sbobj.Groups.Signals(5).XData = [0 20]
      | sbobj.Groups.Signals(5).YData = [1 1]
      | sbobj.Groups.TimeRange = [0 20]
  mu : Outport  Tag=STV Outport  VectorParamsAs1DForOutWhenUnconnected=off
  alpha : Outport  Tag=STV Outport  Port=2  VectorParamsAs1DForOutWhenUnconnected=off
  beta : Outport  Tag=STV Outport  Port=3  VectorParamsAs1DForOutWhenUnconnected=off
  speed brake : Outport  Tag=STV Outport  Port=4
  LandingGear_down : Outport  Tag=STV Outport  Port=5
  wires:
  Demux/5 -> LandingGear_down/1
  Demux/4 -> speed brake/1
  Demux/3 -> beta/1
  Demux/2 -> alpha/1
  Demux/1 -> mu/1
  FromWs/1 -> Demux/1

== system Copy_of_NDI/F-16 Vehicle Systems Model/Pilot commands storehouse/trun(deg)非高攻角 初始高度10000ft 初始速度700ft//s攻角60度 ==
  Demux : Demux  Tag=STV Demux  Outputs=5
      settings: DisplayOption=none
  FromWs : FromWorkspace  Tag=STV FromWs  VariableName=tuvar
      SigBuilderData=|
      | common.afterFinalStr = 'Extrapolate'
      | common.sampleTime = 0
      | dataSet.timeRange = [0 20]
      | dataSet.name = 'Group 5'
      | sbobj.Groups.Name = 'Group 5'
      | sbobj.Groups.Signals(1).Name = 'mu'
      | sbobj.Groups.Signals(1).XData = [0 2 5.5 6 7.2 8.5 10 12 15 20]
      | sbobj.Groups.Signals(1).YData = [0 0 -19.5 -80 -130 -130 -130 -70 -40 -10]
      | sbobj.Groups.Signals(2).Name = 'alpha'
      | sbobj.Groups.Signals(2).XData = [0 5 7.2 7.8 10 12.5 14 20]
      | sbobj.Groups.Signals(2).YData = [7 10 60 60 20 10.68 10 10]
      | sbobj.Groups.Signals(3).Name = 'beta'
      | sbobj.Groups.Signals(3).XData = [0 20]
      | sbobj.Groups.Signals(3).YData = [0 0]
      | sbobj.Groups.Signals(4).Name = 'speed brake'
      | sbobj.Groups.Signals(4).XData = [0 20]
      | sbobj.Groups.Signals(4).YData = [0 0]
      | sbobj.Groups.Signals(5).Name = 'LandingGear_down'
      | sbobj.Groups.Signals(5).XData = [0 20]
      | sbobj.Groups.Signals(5).YData = [1 1]
      | sbobj.Groups.TimeRange = [0 20]
  mu : Outport  Tag=STV Outport  VectorParamsAs1DForOutWhenUnconnected=off
  alpha : Outport  Tag=STV Outport  Port=2  VectorParamsAs1DForOutWhenUnconnected=off
  beta : Outport  Tag=STV Outport  Port=3  VectorParamsAs1DForOutWhenUnconnected=off
  speed brake : Outport  Tag=STV Outport  Port=4
  LandingGear_down : Outport  Tag=STV Outport  Port=5
  wires:
  Demux/5 -> LandingGear_down/1
  Demux/4 -> speed brake/1
  Demux/3 -> beta/1
  Demux/2 -> alpha/1
  Demux/1 -> mu/1
  FromWs/1 -> Demux/1

== system Copy_of_NDI/F-16 Vehicle Systems Model/Pilot commands storehouse/模擬高度15000ft 速度500ft//s ==
  Demux : Demux  Tag=STV Demux  Outputs=5
      settings: DisplayOption=none
  FromWs : FromWorkspace  Tag=STV FromWs  VariableName=tuvar
      SigBuilderData=|
      | common.afterFinalStr = 'Extrapolate'
      | common.sampleTime = 0
      | dataSet.timeRange = [0 20]
      | dataSet.name = 'Group 5'
      | sbobj.Groups.Name = 'Group 5'
      | sbobj.Groups.Signals(1).Name = 'mu'
      | sbobj.Groups.Signals(1).XData = [0 2 20]
      | sbobj.Groups.Signals(1).YData = [0 0 0]
      | sbobj.Groups.Signals(2).Name = 'alpha'
      | sbobj.Groups.Signals(2).XData = [0 0.1 0.9 1.5 2.05 4 5.15 6.05 7.1 7.45 7.72 8.15 9.5 10 10.98 12.02 13.98 20]
      | sbobj.Groups.Signals(2).YData = [7 11 24.5 26 23 16 19 14 14 14 14 14 14 14 12 7 7 7.5]
      | sbobj.Groups.Signals(3).Name = 'beta'
      | sbobj.Groups.Signals(3).XData = [0 20]
      | sbobj.Groups.Signals(3).YData = [0 0]
      | sbobj.Groups.Signals(4).Name = 'speed brake'
      | sbobj.Groups.Signals(4).XData = [0 20]
      | sbobj.Groups.Signals(4).YData = [0 0]
      | sbobj.Groups.Signals(5).Name = 'LandingGear_down'
      | sbobj.Groups.Signals(5).XData = [0 20]
      | sbobj.Groups.Signals(5).YData = [1 1]
      | sbobj.Groups.TimeRange = [0 20]
  mu : Outport  Tag=STV Outport  VectorParamsAs1DForOutWhenUnconnected=off
  alpha : Outport  Tag=STV Outport  Port=2  VectorParamsAs1DForOutWhenUnconnected=off
  beta : Outport  Tag=STV Outport  Port=3  VectorParamsAs1DForOutWhenUnconnected=off
  speed brake : Outport  Tag=STV Outport  Port=4
  LandingGear_down : Outport  Tag=STV Outport  Port=5
  wires:
  FromWs/1 -> Demux/1
  Demux/1 -> mu/1
  Demux/2 -> alpha/1
  Demux/3 -> beta/1
  Demux/4 -> speed brake/1
  Demux/5 -> LandingGear_down/1

== system Copy_of_NDI/F-16 Vehicle Systems Model/Pilot commands storehouse/測試輸入 ==
  Demux : Demux  Tag=STV Demux  Outputs=6
      settings: DisplayOption=none
  FromWs : FromWorkspace  Tag=STV FromWs  VariableName=tuvar
      SigBuilderData=|
      | common.afterFinalStr = 'Extrapolate'
      | common.sampleTime = 0
      | dataSet.timeRange = [0 70]
      | dataSet.name = 'Group 5'
      | sbobj.Groups.Name = 'Group 5'
      | sbobj.Groups.Signals(1).Name = 'thrust'
      | sbobj.Groups.Signals(1).XData = [0 69 70]
      | sbobj.Groups.Signals(1).YData = [10000 10000 9975]
      | sbobj.Groups.Signals(2).Name = 'mu'
      | sbobj.Groups.Signals(2).XData = [0 2 8 10 12 70]
      | sbobj.Groups.Signals(2).YData = [0 0 0 0 0 0]
      | sbobj.Groups.Signals(3).Name = 'alpha'
      | sbobj.Groups.Signals(3).XData = [0 1.4 2 3.7 4.9 5.8 7 8 8.5 9.1 9.9 10.9 13.1 15.25 17.7 19.95 22.7 23.6 30 34.6 39.6 40.35 42.07 48 50 51.35 54.6 56 60 64 70]
      | sbobj.Groups.Signals(3).YData = [7.5 13.5 1.5 2 1.5 1 2.5 3.5 3.5 3.5 3.5 3.5 1.5 1.55 1.8 1.5 1.5 0.9 0.9 0.7 0.4 0.4 0.45 0.23 0.25 0.2 0.2 0.2 0.15 0 0]
      | sbobj.Groups.Signals(4).Name = 'beta'
      | sbobj.Groups.Signals(4).XData = [0 8 70]
      | sbobj.Groups.Signals(4).YData = [0 0 0]
      | sbobj.Groups.Signals(5).Name = 'speed brake'
      | sbobj.Groups.Signals(5).XData = [0 70]
      | sbobj.Groups.Signals(5).YData = [0 0]
      | sbobj.Groups.Signals(6).Name = 'LandingGear_down'
      | sbobj.Groups.Signals(6).XData = [0 70]
      | sbobj.Groups.Signals(6).YData = [1 1]
      | sbobj.Groups.TimeRange = [0 70]
  thrust : Outport  Tag=STV Outport
  mu : Outport  Tag=STV Outport  Port=2  VectorParamsAs1DForOutWhenUnconnected=off
  alpha : Outport  Tag=STV Outport  Port=3  VectorParamsAs1DForOutWhenUnconnected=off
  beta : Outport  Tag=STV Outport  Port=4  VectorParamsAs1DForOutWhenUnconnected=off
  speed brake : Outport  Tag=STV Outport  Port=5
  LandingGear_down : Outport  Tag=STV Outport  Port=6
  wires:
  Demux/6 -> LandingGear_down/1
  Demux/5 -> speed brake/1
  Demux/4 -> beta/1
  Demux/3 -> alpha/1
  Demux/2 -> mu/1
  Demux/1 -> thrust/1
  FromWs/1 -> Demux/1

== system Copy_of_NDI/F-16 Vehicle Systems Model/Pilot commands storehouse/測試輸入(初始高度10000、初始速度500、模擬時間130秒) ==
  Demux : Demux  Tag=STV Demux  Outputs=6
      settings: DisplayOption=none
  FromWs : FromWorkspace  Tag=STV FromWs  VariableName=tuvar
      SigBuilderData=|
      | common.afterFinalStr = 'Extrapolate'
      | common.sampleTime = 0
      | dataSet.timeRange = [0 130]
      | dataSet.name = 'Group 5'
      | sbobj.Groups.Name = 'Group 5'
      | sbobj.Groups.Signals(1).Name = 'thrust'
      | sbobj.Groups.Signals(1).XData = [0 69 71 72.5 74.5 76 78 79.6 81.4 82.6 96.83 130]
      | sbobj.Groups.Signals(1).YData = [10000 10000 9950 9900 9800 9700 9600 9550 9500 9500 9800 9800]
      | sbobj.Groups.Signals(2).Name = 'mu'
      | sbobj.Groups.Signals(2).XData = [0 2 8 10 12 130]
      | sbobj.Groups.Signals(2).YData = [0 0 0 0 0 0]
      | sbobj.Groups.Signals(3).Name = 'alpha'
      | sbobj.Groups.Signals(3).XData = [0 1.4 2 3.7 4.9 5.8 7 8 8.5 9.1 9.9 10.9 13.1 15.25 17.7 19.95 22.7 23.6 30 34.6 39.6 40.35 42.07 48 50 51.35 54.6 56 60 64 130]
      | sbobj.Groups.Signals(3).YData = [7.5 13.5 1.5 2 1.5 1 2.5 3.5 3.5 3.5 3.5 3.5 1.5 1.55 1.8 1.5 1.5 0.9 0.9 0.7 0.4 0.4 0.45 0.23 0.25 0.2 0.2 0.2 0.15 0 0]
      | sbobj.Groups.Signals(4).Name = 'beta'
      | sbobj.Groups.Signals(4).XData = [0 8 130]
      | sbobj.Groups.Signals(4).YData = [0 0 0]
      | sbobj.Groups.Signals(5).Name = 'speed brake'
      | sbobj.Groups.Signals(5).XData = [0 130]
      | sbobj.Groups.Signals(5).YData = [0 0]
      | sbobj.Groups.Signals(6).Name = 'LandingGear_down'
      | sbobj.Groups.Signals(6).XData = [0 130]
      | sbobj.Groups.Signals(6).YData = [1 1]
      | sbobj.Groups.TimeRange = [0 130]
  thrust : Outport  Tag=STV Outport
  mu : Outport  Tag=STV Outport  Port=2  VectorParamsAs1DForOutWhenUnconnected=off
  alpha : Outport  Tag=STV Outport  Port=3  VectorParamsAs1DForOutWhenUnconnected=off
  beta : Outport  Tag=STV Outport  Port=4  VectorParamsAs1DForOutWhenUnconnected=off
  speed brake : Outport  Tag=STV Outport  Port=5
  LandingGear_down : Outport  Tag=STV Outport  Port=6
  wires:
  Demux/6 -> LandingGear_down/1
  Demux/5 -> speed brake/1
  Demux/4 -> beta/1
  Demux/3 -> alpha/1
  Demux/2 -> mu/1
  Demux/1 -> thrust/1
  FromWs/1 -> Demux/1

== system Copy_of_NDI/F-16 Vehicle Systems Model/Pilot commands storehouse/測試輸入(高度10000、速度500、推力10000lb) ==
  Demux : Demux  Tag=STV Demux  Outputs=6
      settings: DisplayOption=none
  FromWs : FromWorkspace  Tag=STV FromWs  VariableName=tuvar
      SigBuilderData=|
      | common.afterFinalStr = 'Extrapolate'
      | common.sampleTime = 0
      | dataSet.timeRange = [0 50]
      | dataSet.name = 'Group 5'
      | sbobj.Groups.Name = 'Group 5'
      | sbobj.Groups.Signals(1).Name = 'thrust'
      | sbobj.Groups.Signals(1).XData = [0 1.8 3.35 5.1 6.7 7.6 8.7 10.45 12.2 13.9 15.55 17.15 18.65 20 21.45 22.7 23.65 25 30 50]
      | sbobj.Groups.Signals(1).YData = [5000 5040 5100 5200 5400 5500 5700 6000 6300 5900 5700 5700 5700 5600 5400 5300 5200 5000 5000 5000]
      | sbobj.Groups.Signals(2).Name = 'mu'
      | sbobj.Groups.Signals(2).XData = [0 2 8 10 12 50]
      | sbobj.Groups.Signals(2).YData = [0 0 0 0 0 0]
      | sbobj.Groups.Signals(3).Name = 'alpha'
      | sbobj.Groups.Signals(3).XData = [0 1.4 2.6 3.7 4.9 5.8 7 8 8.5 9.1 9.9 10.9 13.1 15.25 17.7 19.95 22.7 30 40 50]
      | sbobj.Groups.Signals(3).YData = [7.5 13.5 1.5 2 1.5 1 2.5 1 3 1.5 2 3 2.5 2 2.5 1.5 1.2 0.75 0.6 0.3]
      | sbobj.Groups.Signals(4).Name = 'beta'
      | sbobj.Groups.Signals(4).XData = [0 8 50]
      | sbobj.Groups.Signals(4).YData = [0 0 0]
      | sbobj.Groups.Signals(5).Name = 'speed brake'
      | sbobj.Groups.Signals(5).XData = [0 50]
      | sbobj.Groups.Signals(5).YData = [0 0]
      | sbobj.Groups.Signals(6).Name = 'LandingGear_down'
      | sbobj.Groups.Signals(6).XData = [0 50]
      | sbobj.Groups.Signals(6).YData = [1 1]
      | sbobj.Groups.TimeRange = [0 50]
  thrust : Outport  Tag=STV Outport
  mu : Outport  Tag=STV Outport  Port=2  VectorParamsAs1DForOutWhenUnconnected=off
  alpha : Outport  Tag=STV Outport  Port=3  VectorParamsAs1DForOutWhenUnconnected=off
  beta : Outport  Tag=STV Outport  Port=4  VectorParamsAs1DForOutWhenUnconnected=off
  speed brake : Outport  Tag=STV Outport  Port=5
  LandingGear_down : Outport  Tag=STV Outport  Port=6
  wires:
  Demux/6 -> LandingGear_down/1
  Demux/5 -> speed brake/1
  Demux/4 -> beta/1
  Demux/3 -> alpha/1
  Demux/2 -> mu/1
  Demux/1 -> thrust/1
  FromWs/1 -> Demux/1

== system Copy_of_NDI/F-16 Vehicle Systems Model/Pilot commands storehouse/測試輸入1(高度10000ft 速度530ft//s 推力5000lb) ==
  Demux : Demux  Tag=STV Demux  Outputs=6
      settings: DisplayOption=none
  FromWs : FromWorkspace  Tag=STV FromWs  VariableName=tuvar
      SigBuilderData=|
      | common.afterFinalStr = 'Extrapolate'
      | common.sampleTime = 0
      | dataSet.timeRange = [0 50]
      | dataSet.name = 'Group 5'
      | sbobj.Groups.Name = 'Group 5'
      | sbobj.Groups.Signals(1).Name = 'thrust'
      | sbobj.Groups.Signals(1).XData = [0 2 4 5 6 8 9 10 12 20 25 30 35 40 50]
      | sbobj.Groups.Signals(1).YData = [14400 14300 14300 13800 13100 12000 11500 11100 10700 8000 7600 7100 7000 6800 5700]
      | sbobj.Groups.Signals(2).Name = 'mu'
      | sbobj.Groups.Signals(2).XData = [0 2 8 10 12 50]
      | sbobj.Groups.Signals(2).YData = [0 0 0 0 0 0]
      | sbobj.Groups.Signals(3).Name = 'alpha'
      | sbobj.Groups.Signals(3).XData = [0 1.4 2.6 3.7 4.9 5.8 7 8 9.1 9.95 10.9 30 40 50]
      | sbobj.Groups.Signals(3).YData = [7 6.84 6.76 6.7 6.64 6.6 6.54 6.48 6.42 6.4 6.38 6.36 6.34 6.32]
      | sbobj.Groups.Signals(4).Name = 'beta'
      | sbobj.Groups.Signals(4).XData = [0 8 50]
      | sbobj.Groups.Signals(4).YData = [0 0 0]
      | sbobj.Groups.Signals(5).Name = 'speed brake'
      | sbobj.Groups.Signals(5).XData = [0 50]
      | sbobj.Groups.Signals(5).YData = [0 0]
      | sbobj.Groups.Signals(6).Name = 'LandingGear_down'
      | sbobj.Groups.Signals(6).XData = [0 50]
      | sbobj.Groups.Signals(6).YData = [1 1]
      | sbobj.Groups.TimeRange = [0 50]
  thrust : Outport  Tag=STV Outport
  mu : Outport  Tag=STV Outport  Port=2  VectorParamsAs1DForOutWhenUnconnected=off
  alpha : Outport  Tag=STV Outport  Port=3  VectorParamsAs1DForOutWhenUnconnected=off
  beta : Outport  Tag=STV Outport  Port=4  VectorParamsAs1DForOutWhenUnconnected=off
  speed brake : Outport  Tag=STV Outport  Port=5
  LandingGear_down : Outport  Tag=STV Outport  Port=6
  wires:
  Demux/6 -> LandingGear_down/1
  Demux/5 -> speed brake/1
  Demux/4 -> beta/1
  Demux/3 -> alpha/1
  Demux/2 -> mu/1
  Demux/1 -> thrust/1
  FromWs/1 -> Demux/1

== system Copy_of_NDI/F-16 Vehicle Systems Model/Pilot commands storehouse/落葉飄完整版(碩論6.7) ==
  Demux : Demux  Tag=STV Demux  Outputs=6
      settings: DisplayOption=none
  FromWs : FromWorkspace  Tag=STV FromWs  VariableName=tuvar
      SigBuilderData=|
      | common.afterFinalStr = 'Extrapolate'
      | common.sampleTime = 0
      | dataSet.timeRange = [0 70]
      | dataSet.name = 'Group 5'
      | sbobj.Groups.Name = 'Group 5'
      | sbobj.Groups.Signals(1).Name = 'thrust'
      | sbobj.Groups.Signals(1).XData = [0 2 4 5 6 8 9 10 12 20 25 30 35 40 70]
      | sbobj.Groups.Signals(1).YData = [5100 5100 600 200 200 200 265 3500 3500 3500 6000 15200 15200 10000 10000]
      | sbobj.Groups.Signals(2).Name = 'mu'
      | sbobj.Groups.Signals(2).XData = [0 2 8 10 12 20 30 40 55 67 70]
      | sbobj.Groups.Signals(2).YData = [0 0 0 0 0 90 90 0 80 0 0]
      | sbobj.Groups.Signals(3).Name = 'alpha'
      | sbobj.Groups.Signals(3).XData = [0 1 2 3 10 35 37 60 70]
      | sbobj.Groups.Signals(3).YData = [7 30 31 60 70 70 10 20 20]
      | sbobj.Groups.Signals(4).Name = 'beta'
      | sbobj.Groups.Signals(4).XData = [0 8 70]
      | sbobj.Groups.Signals(4).YData = [0 0 0]
      | sbobj.Groups.Signals(5).Name = 'speed brake'
      | sbobj.Groups.Signals(5).XData = [0 70]
      | sbobj.Groups.Signals(5).YData = [0 0]
      | sbobj.Groups.Signals(6).Name = 'LandingGear_down'
      | sbobj.Groups.Signals(6).XData = [0 70]
      | sbobj.Groups.Signals(6).YData = [1 1]
      | sbobj.Groups.TimeRange = [0 70]
  thrust : Outport  Tag=STV Outport
  mu : Outport  Tag=STV Outport  Port=2  VectorParamsAs1DForOutWhenUnconnected=off
  alpha : Outport  Tag=STV Outport  Port=3  VectorParamsAs1DForOutWhenUnconnected=off
  beta : Outport  Tag=STV Outport  Port=4  VectorParamsAs1DForOutWhenUnconnected=off
  speed brake : Outport  Tag=STV Outport  Port=5
  LandingGear_down : Outport  Tag=STV Outport  Port=6
  wires:
  FromWs/1 -> Demux/1
  Demux/1 -> thrust/1
  Demux/2 -> mu/1
  Demux/3 -> alpha/1
  Demux/4 -> beta/1
  Demux/5 -> speed brake/1
  Demux/6 -> LandingGear_down/1

== system Copy_of_NDI/F-16 Vehicle Systems Model/Pilot commands storehouse/進度報告爬升後模擬測試輸入 (高度10000、速度500、推力10000lb、模擬時間70秒) ==
  Demux : Demux  Tag=STV Demux  Outputs=6
      settings: DisplayOption=none
  FromWs : FromWorkspace  Tag=STV FromWs  VariableName=tuvar
      SigBuilderData=|
      | common.afterFinalStr = 'Extrapolate'
      | common.sampleTime = 0
      | dataSet.timeRange = [0 80]
      | dataSet.name = 'Group 5'
      | sbobj.Groups.Name = 'Group 5'
      | sbobj.Groups.Signals(1).Name = 'thrust'
      | sbobj.Groups.Signals(1).XData = [0 1.8 3.35 5.1 6.7 7.6 8.7 10.45 12.2 13.9 15.55 17.15 18.65 20 21.45 22.7 23.65 25 30 80]
      | sbobj.Groups.Signals(1).YData = [5000 5040 5100 5200 5400 5500 5700 6000 6300 5900 5700 5700 5700 5600 5400 5300 5200 5000 5000 5000]
      | sbobj.Groups.Signals(2).Name = 'mu'
      | sbobj.Groups.Signals(2).XData = [0 2 8 10 12 80]
      | sbobj.Groups.Signals(2).YData = [0 0 0 0 0 0]
      | sbobj.Groups.Signals(3).Name = 'alpha'
      | sbobj.Groups.Signals(3).XData = [0 1.4 2.6 3.7 4.9 5.8 7 8 8.5 9.1 9.9 10.9 15 19.9 22.7 25.55 26.6 27.1 28.45 30 31.3 33 36 39 45 46.2 47 48 49 57.55 64 65.05 66.05 70 80]
      | sbobj.Groups.Signals(3).YData = [7.8 13.8 7.4 2.8 1.8 1.4 1.6 1.8 2 2 2 2 2.05 2.2 1.6 1.6 1.5 1.45 1.2 1.15 1.15 1.05 0.85 0.7 0.6 0.52 0.5 0.45 0.42 0.22 0.15 0.15 0.08 0.06 0.05]
      | sbobj.Groups.Signals(4).Name = 'beta'
      | sbobj.Groups.Signals(4).XData = [0 8 80]
      | sbobj.Groups.Signals(4).YData = [0 0 0]
      | sbobj.Groups.Signals(5).Name = 'speed brake'
      | sbobj.Groups.Signals(5).XData = [0 80]
      | sbobj.Groups.Signals(5).YData = [0 0]
      | sbobj.Groups.Signals(6).Name = 'LandingGear_down'
      | sbobj.Groups.Signals(6).XData = [0 80]
      | sbobj.Groups.Signals(6).YData = [1 1]
      | sbobj.Groups.TimeRange = [0 80]
  thrust : Outport  Tag=STV Outport
  mu : Outport  Tag=STV Outport  Port=2  VectorParamsAs1DForOutWhenUnconnected=off
  alpha : Outport  Tag=STV Outport  Port=3
  beta : Outport  Tag=STV Outport  Port=4  VectorParamsAs1DForOutWhenUnconnected=off
  speed brake : Outport  Tag=STV Outport  Port=5
  LandingGear_down : Outport  Tag=STV Outport  Port=6
  wires:
  FromWs/1 -> Demux/1
  Demux/1 -> thrust/1
  Demux/2 -> mu/1
  Demux/3 -> alpha/1
  Demux/4 -> beta/1
  Demux/5 -> speed brake/1
  Demux/6 -> LandingGear_down/1

== system Copy_of_NDI/F-16 Vehicle Systems Model/Rotation Speed(TVC OFF)OK/If Action Subsystem ==
  pqr command : Inport
  Action Port : ActionPort  ActionPortLabel=if( u1 > 220)
  Out1 : Outport
  wires:
  pqr command/1 -> Out1/1

== system Copy_of_NDI/F-16 Vehicle Systems Model/Rotation Speed(TVC OFF)OK/If Action Subsystem1 ==
  In1 : Inport
  Action Port : ActionPort  ActionPortLabel=elseif(220 >= u1 >= 135)
  Mux1 : Mux  Inputs=3
  Out1 : Outport
  wires:
  In1/1 -> Mux1/3, Mux1/1, Mux1/2
  Mux1/1 -> Out1/1  "pqr dot desire"

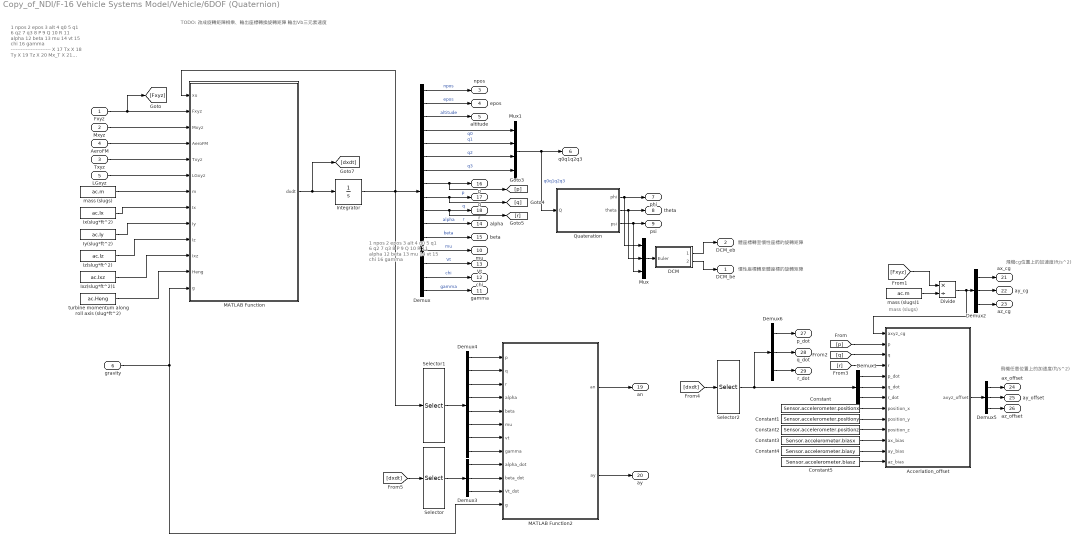
== system Copy_of_NDI/F-16 Vehicle Systems Model/Vehicle/6DOF (Quaternion) ==
  note: TODO: 改成旋轉矩陣相乘、輸出座標轉換旋轉矩陣
      | 輸出Vb三元素速度
  note: 1 npos
      | 2 epos
      | 3 alt
      | 4 q0
      | 5 q1
      | 6 q2
      | 7 q3
      | 8 P
      | 9 Q
      | 10 R
      | 11 alpha
      | 12 beta
      | 13 mu
      | 14 vt
      | 15 chi
      | 16 gamma
      | ------------------------
      | X 17 Tx
      | X 18 Ty
      | X 19 Tz
      | X 20 Mx_T
      | X 21 My_T
      | X 22 Mz_T
      | X 23 T
      | --------------------
      | X 24 ele
      | X 25 ail
      | X 26 rud
      | -------------------
      | X 27 delta_z
      | X 28 delta_y
      | -----------------
      | X 29 qbar
      | -----------------
      | X 30 CXT
      | X 31 CYT
      | X 32 CZT
      | X 33 CLT
      | X 34 CMT
      | X 35 CNT
      | -----------------
      | X 36 lef
  note: 1 npos
      | 2 epos
      | 3 alt
      | 4 q0
      | 5 q1
      | 6 q2
      | 7 q3
      | 8 P
      | 9 Q
      | 10 R
      | 11 alpha
      | 12 beta
      | 13 mu
      | 14 vt
      | 15 chi
      | 16 gamma
  note: 慣性座標轉至體座標的旋轉矩陣
  note: 體座標轉至慣性座標的旋轉矩陣
  note: mass (slugs)
  note: 飛機cg位置上的加速度(ft/s^2)
  note: 飛機任意位置上的加速度(ft/s^2)
  Fxyz : Inport
  Mxyz : Inport  Port=2
  Txyz : Inport  Port=3
  AeroFM : Inport  Port=4
  LGxyz : Inport  Port=5
  gravity : Inport  Port=6
  Accerlation_offset : Subsystem
  Constant : Constant  Value=Sensor.accelerometer.positionx
  Constant1 : Constant  Value=Sensor.accelerometer.positiony
  Constant2 : Constant  Value=Sensor.accelerometer.positionz
  Constant3 : Constant  Value=Sensor.accelerometer.biasx
  Constant4 : Constant  Value=Sensor.accelerometer.biasy
  Constant5 : Constant  Value=Sensor.accelerometer.biasz
  DCM : Subsystem
  Demux : Demux  Outputs=16
      settings: DisplayOption=none
  Demux{1..3,5..6} (5 alike) : Demux  Outputs=3
  Demux4 : Demux  Outputs=8
  Divide : Product  Inputs=*/
  Integrator : Integrator  InitialCondition=state0  ContinuousStateAttributes={'npos', 'epos', 'alt', 'q0', 'q1', 'q2', 'q3', 'P', 'Q', 'R', 'alpha', 'beta', 'mu', 'vt', 'chi', 'gamma'}
  Ix(slug*ft^2) : Constant  Value=ac.Ix
  Ixz(slug*ft^2)1 : Constant  Value=ac.Ixz
  Iy(slug*ft^2) : Constant  Value=ac.Iy
  Iz(slug*ft^2) : Constant  Value=ac.Iz
  MATLAB Function : MATLAB Function  TreatAsAtomicUnit=on
  MATLAB Function2 : MATLAB Function  TreatAsAtomicUnit=on
  Mux : Mux  Inputs=3
  Mux1 : Mux  Inputs=[1,1,1,1]
  Quateration : MATLAB Function  TreatAsAtomicUnit=on
  Selector : Selector  InputPortWidth=16  IndexOptions=Index vector (dialog)  Indices=[11 12 14]  OutputSizes=3
  Selector1 : Selector  InputPortWidth=16  IndexOptions=Index vector (dialog)  Indices=[8:14 16]  OutputSizes=3
  Selector2 : Selector  InputPortWidth=16  IndexOptions=Index vector (dialog)  Indices=[8 9 10]  OutputSizes=3
  mass (slugs) : Constant  Value=ac.m
  mass (slugs)1 : Constant  Value=ac.m
  turbine momentum along roll axis (slug*ft^2) : Constant  Value=ac.Heng
  DCM_be : Outport
  DCM_eb : Outport  Port=2
  npos : Outport  Port=3  VectorParamsAs1DForOutWhenUnconnected=off
  epos : Outport  Port=4  VectorParamsAs1DForOutWhenUnconnected=off
  altitude : Outport  Port=5  VectorParamsAs1DForOutWhenUnconnected=off
  q0q1q2q3 : Outport  Port=6
  phi : Outport  Port=7  VectorParamsAs1DForOutWhenUnconnected=off
  theta : Outport  Port=8  VectorParamsAs1DForOutWhenUnconnected=off
  psi : Outport  Port=9  VectorParamsAs1DForOutWhenUnconnected=off
  mu : Outport  Port=10  VectorParamsAs1DForOutWhenUnconnected=off
  gamma : Outport  Port=11  VectorParamsAs1DForOutWhenUnconnected=off
  chi : Outport  Port=12  VectorParamsAs1DForOutWhenUnconnected=off
  Vt : Outport  Port=13  VectorParamsAs1DForOutWhenUnconnected=off
  alpha : Outport  Port=14  VectorParamsAs1DForOutWhenUnconnected=off
  beta : Outport  Port=15  VectorParamsAs1DForOutWhenUnconnected=off
  p : Outport  Port=16  VectorParamsAs1DForOutWhenUnconnected=off
  q : Outport  Port=17  VectorParamsAs1DForOutWhenUnconnected=off
  r : Outport  Port=18  VectorParamsAs1DForOutWhenUnconnected=off
  an : Outport  Port=19
  ay : Outport  Port=20
  ax_cg : Outport  Port=21
  ay_cg : Outport  Port=22
  az_cg : Outport  Port=23
  ax_offset : Outport  Port=24
  ay_offset : Outport  Port=25
  az_offset : Outport  Port=26
  p_dot : Outport  Port=27
  q_dot : Outport  Port=28
  r_dot : Outport  Port=29
  wires:
  Demux/2 -> epos/1  "epos"
  Demux/3 -> altitude/1  "altitude"
  Integrator/1 -> MATLAB Function/1(xu), Demux/1, Selector1/1
  Demux/1 -> npos/1  "npos"
  Demux/5 -> Mux1/2  "q1"
  Demux/4 -> Mux1/1  "q0"
  Demux/7 -> Mux1/4  "q3"
  Demux/6 -> Mux1/3  "q2"
  Demux/8 -> p/1, [p]  "p"
  Demux/9 -> q/1, [q]  "q"
  Demux/10 -> r/1, [r]  "r"
  Demux/11 -> alpha/1  "alpha"
  Demux/12 -> beta/1  "beta"
  Demux/13 -> mu/1  "mu"
  Demux/14 -> Vt/1  "Vt"
  Demux/15 -> chi/1  "chi"
  Demux/16 -> gamma/1  "gamma"
  Mux1/1 -> q0q1q2q3/1, Quateration/1(Q)  "q0q1q2q3"
  AeroFM/1 -> MATLAB Function/4(AeroFM)
  Mxyz/1 -> MATLAB Function/3(Mxyz)
  Fxyz/1 -> [Fxyz], MATLAB Function/2(Fxyz)
  Txyz/1 -> MATLAB Function/5(Txyz)
  gravity/1 -> MATLAB Function2/12(g), MATLAB Function/13(g)
  Ix(slug*ft^2)/1 -> MATLAB Function/8(Ix)
  Iy(slug*ft^2)/1 -> MATLAB Function/9(Iy)
  Iz(slug*ft^2)/1 -> MATLAB Function/10(Iz)
  Ixz(slug*ft^2)1/1 -> MATLAB Function/11(Ixz)
  turbine momentum along roll axis (slug*ft^2)/1 -> MATLAB Function/12(Heng)
  mass (slugs)/1 -> MATLAB Function/7(m)
  Selector/1 -> Demux3/1
  Demux3/1 -> MATLAB Function2/9(alpha_dot)
  Demux3/2 -> MATLAB Function2/10(beta_dot)
  Demux3/3 -> MATLAB Function2/11(Vt_dot)
  Selector1/1 -> Demux4/1
  Demux4/1 -> MATLAB Function2/1(p)
  Demux4/2 -> MATLAB Function2/2(q)
  Demux4/3 -> MATLAB Function2/3(r)
  Demux4/4 -> MATLAB Function2/4(alpha)
  Demux4/5 -> MATLAB Function2/5(beta)
  Demux4/6 -> MATLAB Function2/6(mu)
  Demux4/7 -> MATLAB Function2/7(vt)
  Demux4/8 -> MATLAB Function2/8(gamma)
  MATLAB Function2/1(an) -> an/1
  MATLAB Function2/2(ay) -> ay/1
  LGxyz/1 -> MATLAB Function/6(LGxyz)
  Quateration/3(psi) -> Mux/3, psi/1
  Quateration/2(theta) -> theta/1, Mux/2
  Quateration/1(phi) -> phi/1, Mux/1
  DCM/1(DCM_eb) -> DCM_eb/1
  DCM/2(DCM_be) -> DCM_be/1
  Constant4/1 -> Accerlation_offset/12(ay_bias)
  Accerlation_offset/1(axyz_offset) -> Demux5/1
  Constant/1 -> Accerlation_offset/8(position_x)
  Selector2/1 -> Demux6/1, Demux1/1
  Demux6/1 -> p_dot/1
  Demux1/2 -> Accerlation_offset/6(q_dot)
  Demux6/2 -> q_dot/1
  Demux5/1 -> ax_offset/1
  Demux5/3 -> az_offset/1
  Demux6/3 -> r_dot/1
  [dxdt] -> Selector2/1
  Demux2/1 -> ax_cg/1
  mass (slugs)1/1 -> Divide/2
  Demux1/1 -> Accerlation_offset/5(p_dot)
  Demux1/3 -> Accerlation_offset/7(r_dot)
  [p] -> Accerlation_offset/2(p)
  [Fxyz] -> Divide/1
  [q] -> Accerlation_offset/3(q)
  Constant1/1 -> Accerlation_offset/9(position_y)
  [r] -> Accerlation_offset/4(r)
  Constant3/1 -> Accerlation_offset/11(ax_bias)
  Constant5/1 -> Accerlation_offset/13(az_bias)
  Demux2/3 -> az_cg/1
  Divide/1 -> Accerlation_offset/1(axyz_cg), Demux2/1
  Constant2/1 -> Accerlation_offset/10(position_z)
  Demux5/2 -> ay_offset/1
  Demux2/2 -> ay_cg/1
  MATLAB Function/1(dxdt) -> [dxdt], Integrator/1
  [dxdt] -> Selector/1
  Mux/1 -> DCM/1(Euler)

== system Copy_of_NDI/F-16 Vehicle Systems Model/Vehicle/Actuators (no roll off)1 ==
  note: 這種建模方式會得到跟順淵不同的結果
  Command : Inport
  "Mach " : Inport  Port=2
  alt : Inport  Port=3
  alpha,beta : Inport  Port=4
  Aileron Saturation : Saturate  UpperLimit=21.5  LowerLimit=-21.5
  Demux1 : Demux  Outputs=6
  Elevator Saturation : Saturate  UpperLimit=25  LowerLimit=-25
  Engine block : Subsystem
  Fcn : Fcn  Expr=u(1)*cos(u(2))*cos(u(3))
  Integrator (degrees) : Integrator  Commented=through  InitialCondition=0.015206  UpperSaturationLimit=30  LowerSaturationLimit=-30
  Integrator (degrees)1 : Integrator  Commented=through  UpperSaturationLimit=30  LowerSaturationLimit=-30
  Integrator (degrees)2 : Integrator  Commented=on  UpperSaturationLimit=30  LowerSaturationLimit=-30
  Integrator(degrees) : Integrator  Commented=on  InitialCondition=-0.051516  UpperSaturationLimit=21.5  LowerSaturationLimit=-21.5
  "Integrator(degrees) " : Integrator  Commented=on  InitialCondition=-4.2454  UpperSaturationLimit=25  LowerSaturationLimit=-25
  Mux1 : Mux  Inputs=2
  Mux9 : Mux  Inputs=6
  Rate Limiter : RateLimiter  RisingSlewLimit=+60  FallingSlewLimit=-60  SampleTimeMode=inherited
  Rate Limiter1 : RateLimiter  RisingSlewLimit=+80  FallingSlewLimit=-80  SampleTimeMode=inherited
  Rate Limiter2 : RateLimiter  RisingSlewLimit=+120  FallingSlewLimit=-120  SampleTimeMode=inherited
  Rate Limiter3 : RateLimiter  RisingSlewLimit=+60  FallingSlewLimit=-60  SampleTimeMode=inherited
  Rate Limiter4 : RateLimiter  RisingSlewLimit=+60  FallingSlewLimit=-60  SampleTimeMode=inherited
  Rudder Saturation : Saturate  UpperLimit=30  LowerLimit=-30
  Saturation : Saturate  UpperLimit=50000  LowerLimit=0
  Saturation Dynamic : simulink/Discontinuities/Saturation Dynamic  OutMin=[]  OutMax=[]  OutDataTypeStr=Inherit: Same as second input  OutDataType=fixdt(1, 16)  OutScaling=2^-10  DoSatur=off
  TVC_Y Saturation : Saturate  UpperLimit=15  LowerLimit=-15
  TVC_Z Saturation : Saturate  UpperLimit=15  LowerLimit=-15
  Transfer Fcn{,1..4} (5 alike) : TransferFcn  Numerator=[20.202]  Denominator=[1 20.202]
  r2d2 : Gain  Gain=-1  SaturateOnIntegerOverflow=on  OutDataTypeStr=Inherit: Same as input  ParamDataTypeStr=Inherit: Same as input
  Actuator : Outport  VectorParamsAs1DForOutWhenUnconnected=off
  wires:
  Mux9/1 -> Actuator/1
  Command/1 -> Demux1/1
  Transfer Fcn/1 -> Mux9/2  "elevator"
  Transfer Fcn1/1 -> Mux9/3  "Aileron"
  Transfer Fcn2/1 -> Mux9/4  "Rudder"
  Saturation Dynamic/1 -> Mux9/1  "thrust"
  Transfer Fcn4/1 -> Mux9/6  "yaw vector"
  Transfer Fcn3/1 -> Mux9/5  "pitch vector"
  r2d2/1 -> Saturation/1
  alt/1 -> r2d2/1
  Demux1/1 -> Saturation Dynamic/2
  "Mach "/1 -> Mux1/1
  alpha,beta/1 -> Mux1/2
  Mux1/1 -> Fcn/1
  Fcn/1 -> Engine block/1(Mach)
  Saturation/1 -> Engine block/2(Attitude)
  Engine block/2(T_min) -> Saturation Dynamic/3
  Engine block/1(T_max) -> Saturation Dynamic/1
  Demux1/2 -> Elevator Saturation/1
  Elevator Saturation/1 -> Rate Limiter/1
  Demux1/3 -> Aileron Saturation/1
  Aileron Saturation/1 -> Rate Limiter1/1
  Demux1/4 -> Rudder Saturation/1
  Rudder Saturation/1 -> Rate Limiter2/1
  Demux1/5 -> TVC_Z Saturation/1
  TVC_Z Saturation/1 -> Rate Limiter3/1
  Demux1/6 -> TVC_Y Saturation/1
  TVC_Y Saturation/1 -> Rate Limiter4/1
  Rate Limiter/1 -> Transfer Fcn/1
  Rate Limiter1/1 -> Transfer Fcn1/1
  Rate Limiter2/1 -> Transfer Fcn2/1
  Rate Limiter3/1 -> Transfer Fcn3/1
  Rate Limiter4/1 -> Transfer Fcn4/1

== system Copy_of_NDI/F-16 Vehicle Systems Model/Vehicle/Aerodynamics ==
  note: TODO: 這全部源自PlantData(物理系統)，不用感測器
  note: TODO: 這攻角、速度 來自感測器、AeroData System
  note: X
      | Y
      | Z
      | L
      | M
      | N
  note: 攻角 $\alpha$ 限制 -20 ~ 90度
      | 側滑角 $\beta$ 限制 -30 ~ 30 度
      | 馬赫數限制 0.1 ~ 0.6 度
  fcs_cmd : Inport
  " SB (deg)" : Inport  Port=2
  In Bus Element7 : Inport  Port=3  PortName=EnvData  Element=Pressure
  In Bus Element8 : Inport  Port=3  PortName=EnvData  Element=AirDensity
  In Bus Element9 : Inport  Port=3  PortName=EnvData  Element=qbar
  In Bus Element : Inport  Port=4  PortName=PlantData  Element=p
  In Bus Element1 : Inport  Port=4  PortName=PlantData  Element=q
  In Bus Element2 : Inport  Port=4  PortName=PlantData  Element=r
  In Bus Element3 : Inport  Port=4  PortName=PlantData  Element=alpha
  In Bus Element10 : Inport  Port=4  PortName=PlantData  Element=alpha
  In Bus Element4 : Inport  Port=4  PortName=PlantData  Element=beta
  In Bus Element6 : Inport  Port=4  PortName=PlantData  Element=Vt
  In Bus Element5 : Inport  Port=4  PortName=PlantData  Element=Vt
  Aerofynamic Coefficients : Subsystem
  AirframeActuators (no roll off) : Subsystem
  Angle Conversion1 : aerolibconvert2/Angle Conversion  IU=rad  OU=deg
  Angle Conversion2 : aerolibconvert2/Angle Conversion  IU=rad  OU=deg
  Angle Conversion3 : aerolibconvert2/Angle Conversion  Commented=on  IU=rad  OU=deg
  Bus Creator : BusCreator  Inputs=7
  Bus Selector : BusSelector  OutputSignals=right Aileron_deg,left Aileron_deg,right Elevator_deg,left Elevator_deg,Rudder_deg,LEF_deg
  Bus Selector1 : BusSelector  OutputSignals=right Aileron_deg,left Aileron_deg,right Elevator_deg,left Elevator_deg,Rudder_deg,LEF_deg
  Bus Selector2 : BusSelector  Commented=on  OutputSignals=LEF_deg
  Cbar(ft)1 : Constant  Value=ac.cbar
  Goto2 : Goto  Commented=on  GotoTag=LEF_deg
  Ground : Ground
  Leading Edge Flap : Subsystem  Commented=on
  Mux1 : Mux  Inputs=3
  Mux2 : Mux
  Product{6,9..14} (7 alike) : Product
  Sref(ft^2) : Constant  Value=ac.S
  Terminator{,1..3} (4 alike) : Terminator
  Velocity Conversion : aerolibconvert2/Velocity Conversion  Commented=on  IU=ft/s  OU=m/s
  b(ft)1 : Constant  Value=ac.b
  FM : Outport
  Bus Element Out : Outport  Port=2  PortName=ActSensor_Out
  wires:
  " SB (deg)"/1 -> Aerofynamic Coefficients/9(SB (deg)), Bus Creator/7  "SB_deg"
  In Bus Element1/1 -> Aerofynamic Coefficients/12(q)
  In Bus Element/1 -> Aerofynamic Coefficients/11(p)
  Angle Conversion2/1 -> Aerofynamic Coefficients/2(beta (deg))
  Angle Conversion1/1 -> Aerofynamic Coefficients/1(alpha (deg))
  In Bus Element2/1 -> Aerofynamic Coefficients/13(r)
  Ground/1 -> Aerofynamic Coefficients/15(h_AGL), Aerofynamic Coefficients/14(GearAngle)
  Mux1/1 -> Product9/2
  [qbar_S] -> Product9/1
  Aerofynamic Coefficients/6(Cn_T) -> Product14/2
  Aerofynamic Coefficients/5(Cm_T) -> Product12/2
  [qbar_S_cbar] -> Product12/1  "qbar_S_cbar"
  Aerofynamic Coefficients/4(Cl_T) -> Product13/2
  [qbar_S_b] -> Product13/1, Product14/1  "qbar_S_b"
  Aerofynamic Coefficients/1(CX_T) -> Mux1/1
  Aerofynamic Coefficients/2(CY_T) -> Mux1/2
  Aerofynamic Coefficients/3(CZ_T) -> Mux1/3
  Product13/1 -> Mux2/2
  Product12/1 -> Mux2/3
  Product14/1 -> Mux2/4
  Product9/1 -> Mux2/1
  Mux2/1 -> FM/1
  Sref(ft^2)/1 -> Product6/2
  b(ft)1/1 -> Product11/2  "b"
  Product11/1 -> [qbar_S_b]
  Product10/1 -> [qbar_S_cbar]
  Cbar(ft)1/1 -> Product10/2  "cbar"
  In Bus Element9/1 -> Product6/1  "qbar"
  Product6/1 -> Product11/1, Product10/1, [qbar_S]  "qbar_S"
  Leading Edge Flap/2(ActPositions) -> Goto2/1
  Velocity Conversion/1 -> Leading Edge Flap/1(vt (m/s))  "vt (m/s)"
  In Bus Element6/1 -> Aerofynamic Coefficients/10(vt (ft/s))
  In Bus Element8/1 -> Terminator1/1
  In Bus Element7/1 -> Terminator2/1
  AirframeActuators (no roll off)/1(ActPositions) -> Bus Selector/1
  fcs_cmd/1 -> AirframeActuators (no roll off)/1(fcs_cmd)
  In Bus Element3/1 -> Angle Conversion1/1
  In Bus Element4/1 -> Angle Conversion2/1
  In Bus Element5/1 -> Terminator/1  "vt (ft/s)"
  AirframeActuators (no roll off)/2(ActSensor_Out) -> Bus Selector1/1
  Bus Creator/1 -> Bus Element Out/1
  In Bus Element10/1 -> Terminator3/1
  Angle Conversion3/1 -> Leading Edge Flap/4(alpha (deg))
  Leading Edge Flap/1(ActSensor_Out) -> Bus Selector2/1
  Bus Selector1/1 -> Bus Creator/1  "<right Aileron_deg>"
  Bus Selector1/2 -> Bus Creator/2  "<left Aileron_deg>"
  Bus Selector1/3 -> Bus Creator/3  "<right Elevator_deg>"
  Bus Selector1/4 -> Bus Creator/4  "<left Elevator_deg>"
  Bus Selector1/5 -> Bus Creator/5  "<Rudder_deg>"
  Bus Selector1/6 -> Bus Creator/6  "<LEF_deg>"
  Bus Selector/1 -> Aerofynamic Coefficients/3(right alieron (deg))  "<right Aileron_deg>"
  Bus Selector/2 -> Aerofynamic Coefficients/4(left aileron (deg))  "<left Aileron_deg>"
  Bus Selector/5 -> Aerofynamic Coefficients/7(rudder (deg))  "<Rudder_deg>"
  Bus Selector/6 -> Aerofynamic Coefficients/8(LEF (deg))  "<LEF_deg>"
  Bus Selector/4 -> Aerofynamic Coefficients/6(left elevator (deg))  "<left Elevator_deg>"
  Bus Selector/3 -> Aerofynamic Coefficients/5(right elevator (deg))  "<right Elevator_deg>"

== system Copy_of_NDI/F-16 Vehicle Systems Model/Vehicle/Gravity Force ==
  note: 轉成行向量(column vector)
  note: 註：重力不會對飛機產生力矩，
      | 因為重力永遠作用在飛機重心上，
      | 力臂=0，所以力矩=0
  DCM_be : Inport
  In Bus Element : Inport  Port=2  PortName=EnvData  Element=g
  Gravity in Earth Axis : Gain  Gain=ac.m
  Reshape : Reshape  OutputDimensionality=Column vector (2-D)
  To Body Axes : Product  Multiplication=Matrix(*)
  Fgrav : Outport
  wires:
  In Bus Element/1 -> Gravity in Earth Axis/1
  To Body Axes/1 -> Fgrav/1
  DCM_be/1 -> To Body Axes/1
  Gravity in Earth Axis/1 -> Reshape/1
  Reshape/1 -> To Body Axes/2

== system Copy_of_NDI/F-16 Vehicle Systems Model/Vehicle/LandingGear GroundReaction ==
  note: 定義：
      | 慣性座標+Z軸朝上
      | 體座標+Z軸朝下
  note: 詹庭宇:
      | 此起落架模組源自MATLAB Simulink Example:HL-20
      | 我有做
      | 1.正負號的訂正
      | 2.拿掉/忽略輪胎側向力
  note: 詹庭宇:拿掉/忽略輪胎側向力模型，Fy=0
  LG_cmd : Inport
  In Bus Element4 : Inport  Port=2  PortName=EnvData  Element=hground
  In Bus Element5 : Inport  Port=2  PortName=EnvData  Element=hground
  In Bus Element6 : Inport  Port=2  PortName=EnvData  Element=hground
  In Bus Element3 : Inport  Port=3  PortName=PlantData
  In Bus Element1 : Inport  Port=3  PortName=PlantData
  In Bus Element2 : Inport  Port=3  PortName=PlantData
  Enable : EnablePort
  Demux : Demux  Outputs=3
  L Main Gear Geometry Forces and Moments : Subsystem  TreatAsAtomicUnit=on
  LeftMain : Selector  NumberOfDimensions=2  InputPortWidth=3  IndexOptions=Select all,Index vector (dialog)  Indices=-1,1  OutputSizes=1
  Nose : Selector  NumberOfDimensions=2  InputPortWidth=3  IndexOptions=Select all,Index vector (dialog)  Indices=-1,3  OutputSizes=1
  Nose Gear Geometry Forces and Moments : Subsystem  TreatAsAtomicUnit=on
  Pos_full_extend_ft Rows are X,Y,Z;cols are Left,Right,Nose gear Measured from CG in fts : Constant  Value=[-1.8405,-1.8405,9.9132 ; -3.8753,3.8753,0 ; 5.9161,5.9161, 6.2905]
  R Main Gear Geometry Forces and Moments : Subsystem  TreatAsAtomicUnit=on
  RightMain : Selector  NumberOfDimensions=2  InputPortWidth=3  IndexOptions=Select all,Index vector (dialog)  Indices=-1,2  OutputSizes=1
  Sum2 : Sum  Inputs=+++  InputSameDT=on  SaturateOnIntegerOverflow=on  OutDataTypeStr=Inherit: Same as first input
  FM : Outport
  Out Bus Element3 : Outport  Port=2  VectorParamsAs1DForOutWhenUnconnected=off  PortName=LGData  Element=Nose_WOW
  Out Bus Element4 : Outport  Port=2  VectorParamsAs1DForOutWhenUnconnected=off  PortName=LGData  Element=Nose_GearCmprs
  Out Bus Element5 : Outport  Port=2  VectorParamsAs1DForOutWhenUnconnected=off  PortName=LGData  Element=Nose_LG_down
  Out Bus Element6 : Outport  Port=2  VectorParamsAs1DForOutWhenUnconnected=off  PortName=LGData  Element=LeftMain_WOW
  Out Bus Element7 : Outport  Port=2  VectorParamsAs1DForOutWhenUnconnected=off  PortName=LGData  Element=LeftMain_GearCmprs
  Out Bus Element8 : Outport  Port=2  VectorParamsAs1DForOutWhenUnconnected=off  PortName=LGData  Element=LeftMain_LG_down
  Out Bus Element9 : Outport  Port=2  VectorParamsAs1DForOutWhenUnconnected=off  PortName=LGData  Element=RightMain_WOW
  Out Bus Element10 : Outport  Port=2  VectorParamsAs1DForOutWhenUnconnected=off  PortName=LGData  Element=RightMain_GearCmprs
  Out Bus Element11 : Outport  Port=2  VectorParamsAs1DForOutWhenUnconnected=off  PortName=LGData  Element=RightMain_LG_down
  wires:
  In Bus Element4/1 -> L Main Gear Geometry Forces and Moments/1(ground_z_ft)
  In Bus Element3/1 -> L Main Gear Geometry Forces and Moments/2(plant)
  In Bus Element1/1 -> R Main Gear Geometry Forces and Moments/2(plant)
  In Bus Element2/1 -> Nose Gear Geometry Forces and Moments/2(plant)
  R Main Gear Geometry Forces and Moments/1(FM) -> Sum2/2
  L Main Gear Geometry Forces and Moments/1(FM) -> Sum2/1
  R Main Gear Geometry Forces and Moments/3(GearCmprs) -> Out Bus Element10/1
  R Main Gear Geometry Forces and Moments/2(WOW) -> Out Bus Element9/1
  L Main Gear Geometry Forces and Moments/2(WOW) -> Out Bus Element6/1
  L Main Gear Geometry Forces and Moments/3(GearCmprs) -> Out Bus Element7/1
  RightMain/1 -> R Main Gear Geometry Forces and Moments/3(GearLoc)
  Nose/1 -> Nose Gear Geometry Forces and Moments/3(GearLoc)
  Pos_full_extend_ft Rows are X,Y,Z;cols are Left,Right,Nose gear Measured from CG in fts/1 -> LeftMain/1, Nose/1, RightMain/1
  Nose Gear Geometry Forces and Moments/1(FM) -> Sum2/3
  Nose Gear Geometry Forces and Moments/2(WOW) -> Out Bus Element3/1
  Nose Gear Geometry Forces and Moments/3(GearCmprs) -> Out Bus Element4/1
  Sum2/1 -> FM/1
  LeftMain/1 -> L Main Gear Geometry Forces and Moments/3(GearLoc)
  LG_cmd/1 -> Demux/1
  Demux/1 -> Out Bus Element5/1
  Demux/2 -> Out Bus Element11/1
  Demux/3 -> Out Bus Element8/1
  In Bus Element5/1 -> R Main Gear Geometry Forces and Moments/1(ground_z_ft)
  In Bus Element6/1 -> Nose Gear Geometry Forces and Moments/1(ground_z_ft)

== system Copy_of_NDI/F-16 Vehicle Systems Model/Vehicle/Propulsion ==
  note: 繞"固定座標旋轉"旋轉(外在旋轉extrinsic rotation)
  note: Thrust Vector Nozzle Module 向量噴嘴模組
  note: Commands_TVC_rY_pitch_deg
      | Commands_TVC_rZ_yaw_deg
      | Commands_TVC_lY_pitch_deg
      | Commands_TVC_lZ_yaw_deg
  note: Inlet 進氣道
  note: 高度限制 0 ~ 50000 ft
      | 馬赫數限制 0 ~ 1 馬赫
  Bus Element In2 : Inport  PortName=fadec_cmd
  In Bus Element3 : Inport  PortName=fadec_cmd  Element=thrust
  In Bus Element1 : Inport  Port=2  PortName=EnvData  Element=Mach
  Bus Element In1 : Inport  Port=3  PortName=PlantData  Element=beta
  Bus Element In : Inport  Port=3  PortName=PlantData  Element=alpha
  In Bus Element : Inport  Port=3  PortName=PlantData  Element=altitude
  Actuators : Subsystem
  Afterburning Turbofan Jet Engine : Subsystem
  Cos : Trigonometry  Operator=cos
  Cos1 : Trigonometry  Operator=cos
  Gain1 : Gain  Gain=0.5
  IC1 : InitialCondition  Commented=through  Value=IC.thrust_lbf
  Product : Product  Inputs=3
  Thrust Vector Nozzle ZY1 : Subsystem
  nozzle position1 : Constant  Value=ac.lt1
  nozzle position2 : Constant  Value=ac.mt
  r2d1 : Gain  Gain=-1  SaturateOnIntegerOverflow=on  OutDataTypeStr=Inherit: Same as input  ParamDataTypeStr=Inherit: Same as input
  FM : Outport
  Bus Element Out : Outport  Port=2  PortName=ActSensor_Out
  Bus Element Out1 : Outport  Port=3  PortName=PropData  Element=Tx
  Bus Element Out2 : Outport  Port=3  PortName=PropData  Element=Ty
  Bus Element Out3 : Outport  Port=3  PortName=PropData  Element=Tz
  Bus Element Out4 : Outport  Port=3  PortName=PropData  Element=T
  Bus Element Out5 : Outport  Port=3  PortName=PropData  Element=engine_state
  wires:
  Actuators/2(ActSensor_Out) -> Bus Element Out/1
  nozzle position1/1 -> Thrust Vector Nozzle ZY1/3(" lt1")
  Actuators/1(ActPositions) -> Thrust Vector Nozzle ZY1/2(Actuator (deg))
  Thrust Vector Nozzle ZY1/1(FM) -> FM/1
  Product/1 -> Afterburning Turbofan Jet Engine/1(Mach)
  r2d1/1 -> Afterburning Turbofan Jet Engine/2(H (ft))
  Cos/1 -> Product/2
  Bus Element In1/1 -> Cos1/1  "beta (rad)"
  In Bus Element1/1 -> Product/1
  Cos1/1 -> Product/3
  Bus Element In/1 -> Cos/1  "alpha (rad)"
  In Bus Element/1 -> r2d1/1
  Bus Element In2/1 -> Actuators/1(Commands)
  Thrust Vector Nozzle ZY1/2(Tx) -> Bus Element Out1/1
  Thrust Vector Nozzle ZY1/3(Ty) -> Bus Element Out2/1
  Thrust Vector Nozzle ZY1/4(Tz) -> Bus Element Out3/1
  nozzle position2/1 -> Thrust Vector Nozzle ZY1/4(" mt")
  IC1/1 -> Gain1/1, Bus Element Out4/1  "thrust"
  Afterburning Turbofan Jet Engine/1(T (lbf)) -> IC1/1  "thrust"
  Afterburning Turbofan Jet Engine/2(engine_state) -> Bus Element Out5/1
  In Bus Element3/1 -> Afterburning Turbofan Jet Engine/3(Tc (lbf))  "Commands_Tc"
  Gain1/1 -> Thrust Vector Nozzle ZY1/1(T1)  "thrust"
